simulink library "MCHP_Blockset"  (Simulink 7.5)
settings: Solver=ode45  SolverMode=SingleTasking  StartTime=0.0  StopTime=10.0  RelTol=1e-3
InitFcn:
  | disp('MCHP_Blockset_Library_InitFunction');
undefined symbols (not defined in the file): A0, A2, AD0, AVdd, B1, B5, B9, C10, C2, CMP2A, CMP3A, CMP4A, EXTREF1, EXTREF2, gcbh, MaxPer, MCHP_ACC_SAMx_Callback, MCHP_ADC_Callback, MCHP_ADC_HighSpeed_SAR_Callback, MCHP_ADC_HighSpeed_SAR_dsPIC_Callback, MCHP_ADC_SAME5x_Callback, MCHP_AFEC_SAM7x_Callback, MCHP_BUS_I2C_MASTER_callback, MCHP_BUS_SPI_callback, MCHP_C_function_Call_callback, MCHP_CN_Callback, MCHP_COMPARATOR1_callback, MCHP_CompilerOptimisation_Callback, MCHP_DACC_SAMx_Callback, MCHP_Digital_Input_Callback, MCHP_Digital_Output_Read_Callback, MCHP_Digital_Output_Write_Callback, MCHP_Fun, MCHP_HighSpeed_AnalogComparator_Callback, MCHP_IC_Callback, MCHP_IdleTask_Callback, MCHP_Interrupt_Callback, MCHP_Master_Callback, MCHP_MCPWM_Callback, MCHP_MCU_LOAD_Callback, MCHP_MCU_OVERLOAD_Callback, MCHP_MSI_Callback, MCHP_OC_HW_Callback, MCHP_OC_SW_Callback, MCHP_OP_AMP_Callback, MCHP_OrderInOut, MCHP_PDEC_Callback, MCHP_PGA_Callback, MCHP_PWM_Callback, MCHP_PWM_HighSpeed_Override_Callback, MCHP_PWM_HS_FEP_Callback, MCHP_PWM_SAM7x_Callback, MCHP_PWM_SAM7x_Override_Callback, MCHP_QDEC_SAMx_Callback, MCHP_QEI_Callback, MCHP_Scheduler_Options_Callback, MCHP_SECONDARY_CORE_Callback, MCHP_Tasks_State_Callback, MCHP_TCC_PWM_Callback, MCHP_TIMER_Config_Callback ... (+18)
libraries: MCHP_Blockset x2
(part 2 of 9)

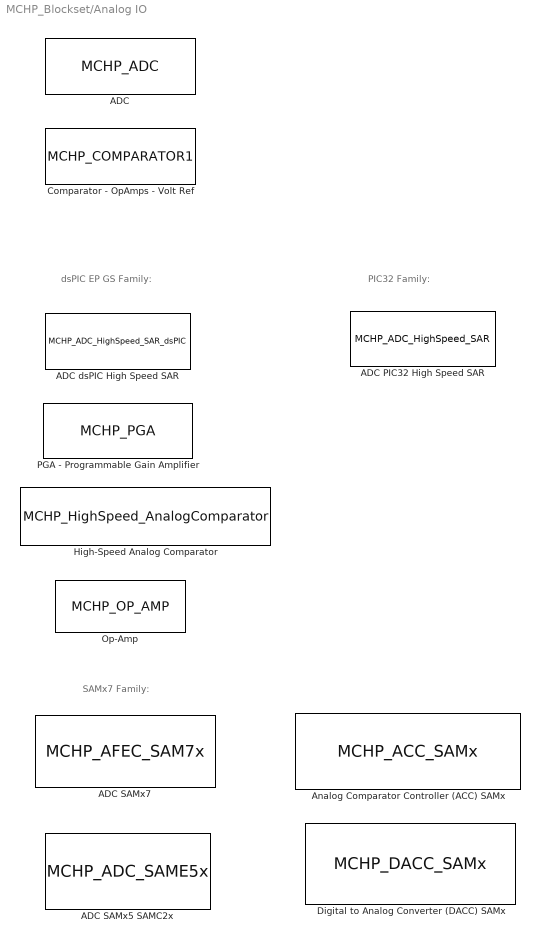
== system MCHP_Blockset/Analog IO ==
  note: dsPIC EP GS Family:
  note: PIC32 Family:
  note: SAMx7 Family:
  ADC : S-Function  Priority=5  InitFcn=MCHP_ADC_Callback(gcbh,'InitFcn');  FunctionName=MCHP_ADC  Parameters=SampleTime,[],MCHP_ADC_Callback(gcbh,'OutputType'),[],MCHP_ADC_Callback(gcbh,'OutputSize')  EnableBusSupport=off  mask{ADC_REF=1, Mode=10 bits (allows exact simultaneous sampling), FORM=0000 dddd dddd dddd ==> Unsigned integer, ADC_R=< 5    kOhm, nSAMPLECHANNELS=CH0 only, nSAMPLECHANNELS_12bits=CH0 only, SIMULTANEOUS=Simultaneously on all Channels, ADxCSS=[1 2], MUXA_CH0N=off, MUXA_CH123=Dynamic Options, MUXA_CH123_TXT=0, MUXB_CH0=AN1, MUXB_CH0N=on, MUXB_CH123=Dynamic Options, MUXB_CH123_TXT=0, SequenceRepeat=1, SequenceTiming=are done as fast as possible at end of previous time step, SSRC_SSRCG=Dynamic Options, SSRC_SSRCG_TXT=0, Update_BlockOutput=After all trig and conversion sequence, Trig_TimeStep=with each update of the ADC block output, ADC_DMA_CHANNEL=Use Interrupt instead of DMA, SampleTime=-1, Info=, MCHP_PORT=, MCHP_MASTERLINK=Testing_MasterBlock/Microchip Master, ADC_TIMING=0}
      mask prompts: ADC_REF "ADC"; FORM "Output Format"; ADC_R "Input Impedance"; nSAMPLECHANNELS "Sample and Hold Capacitor, and Sequences :"; nSAMPLECHANNELS_12bits "1 or 2 Sequences"; SIMULTANEOUS "Sampling happend:"; ADxCSS "CH0 Sequential Sampling, ex: [0 1 4 6] for AN0, AN1, AN4 and AN6"; MUXA_CH0N "Substract AN1 to CH0 (CH0 - AN1)"; MUXA_CH123 "CH1 : CH2 : CH3"; MUXB_CH0 "CH0 (B)"; MUXB_CH0N "Substract AN1 to CH0 (CH0 - AN1) (B)"; MUXB_CH123 "CH1 : CH2 : CH3 (B)"; SequenceRepeat "Repeat conversion sequence xx times"; SequenceTiming "Samples and Conversions"; SSRC_SSRCG "Trigger"; SSRC_SSRCG_TXT "Trigger SSRC_SSRCG value"; Update_BlockOutput "Update block output"; Trig_TimeStep "Trig Time Step"; ADC_DMA_CHANNEL "DMA"; SampleTime "Block Sample Time"
      mask init:
      | MCHP_ADC_Callback(gcbh,'INITIALISATION');
      settings: CopyFcn=MCHP_ADC_Callback(gcbh,'INITIALISATION');  PreSaveFcn=MCHP_ADC_Callback(gcbh,'InitFcn');MCHP_Fun.PreSaveFcn_DynamicOptions(gcbh);  OpenFcn=MCHP_ADC_Callback(gcbh,'OPEN');
      mask StyleString: popup(1),popup(10 bits (allows exact simultaneous sampling)|12 bits),popup(0000 dddd dddd dddd ==> Unsigned integer|ssss sddd dddd dddd ==> Signed integer|dddd dddd dddd 0000 ==> Unsigned fractional|sddd dddd dddd 0000  ==> Signed fractional),popup(< 100 Ohm|< 200 Ohm|< 500 Ohm|< 1    kOhm|< 2    kOhm|< 5    kOhm|< 10   kOhm|< 20   kOhm|< 50   kOhm|< 100  kOhm|< 200  kOhm|< 500  kOhm|< 1000 kOhm|max sampling time),popup(CH0 only|CH0 : CH1|CH0 : CH1 : CH2 : CH3|CH0 two sequences (A & B)|CH0 : CH1 two sequences (A & B)|CH0 : CH1 : CH2 : CH3 two seq (A & B)),popup(CH0 only|CH0 two sequences (A & B)),popup(Simultaneously on all Channels|in Sequence),edit,checkbox,popup(Dynamic Options),edit,popup(AN0|AN1|AN2|AN3|AN4|AN5|AN6|AN7|AN8|AN9|AN10|AN11|AN12|AN13|AN14|AN15|AN16|AN17|AN18|AN19|AN20|AN21|AN22|AN23|AN24|AN25|AN26|AN27|AN28|AN29|AN30|AN31|AN32|AN33|AN34|AN35|AN36|AN37|AN38|AN39|AN40|AN41|AN42|AN43|AN44|AN45|AN46|AN47|AN48|AN49|AN50|AN51|AN52|AN53|AN54|AN55|AN56|AN57|AN58|AN59|AN60|AN61|AN62|AN63|AN64|AN65|AN66|AN67|AN68|AN69|AN70|AN71|AN72|AN73|AN74|AN75|AN76|AN77|AN78|AN79|AN80|AN81|AN82|AN83|AN84|AN85|AN86|AN87|AN88|AN89|AN90|AN91|AN92|AN93|AN94|AN95|AN96|AN97|AN98|AN99|OA1|OA2|OA3|OA4|OA4),checkbox,popup(Dynamic Options),edit,edit,popup(are done as fast as possible at end of previous time step|are done as fast as possible ; triggered by user define source|are stretcheded to fit exactly previous time step|are continuously sampling as fast as possible),popup(Dynamic Options),edit,popup(After all trig and conversion sequence|After each trig and conversion sequence),popup(with each update of the ADC block output|not synchronised with ADC [timer based...]),popup(Use Interrupt instead of DMA|use DMA Channel 0|use DMA Channel 1|use DMA Channel 2|use DMA Channel 3|use DMA Channel 4|use DMA Channel 5|use DMA Channel 6|use DMA Channel 7|use DMA Channel 8|use DMA Channel 9|use DMA Channel 10|use DMA Channel 11|use DMA Channel 12|use DMA Channel 13|use DMA Channel 14|use DMA Channel 15),edit,edit,edit,edit,edit
      mask CallbackString: |MCHP_ADC_Callback(gcbh,'Mode');||MCHP_ADC_Callback(gcbh,'ADC_R');|MCHP_ADC_Callback(gcbh,'nSAMPLECHANNELS');|MCHP_ADC_Callback(gcbh,'nSAMPLECHANNELS_12bits');|MCHP_ADC_Callback(gcbh,'SIMULTANEOUS');|MCHP_ADC_Callback(gcbh,'ADxCSS');|MCHP_ADC_Callback(gcbh,'MUXA_CH0N');|MCHP_ADC_Callback(gcbh,'MUXA_CH123');||MCHP_ADC_Callback(gcbh,'MUXA_CH123');|MCHP_ADC_Callback(gcbh,'MUXA_CH123');||||MCHP_ADC_Callback(gcbh,'SequenceTiming');|||MCHP_ADC_Callback(gcbh,'Update_BlockOutput');|||||||
      mask TabNameString: ADC,ADC,ADC,ADC,ADC,ADC,ADC,ADC,ADC,ADC,ADC,ADC,ADC,ADC,ADC,ADC,Trig and Time Step,Trig and Time Step,Trig and Time Step,Trig and Time Step,Trig and Time Step,ADC,ADC,ADC,ADC,ADC,ADC
      mask Display:
      | MCHP_DrawLogo;
      | fprintf('ADC 1');
      | port_label('output',1,'AN1');
      | port_label('output',2,'AN2');
  ADC PIC32 High Speed SAR : S-Function  InitFcn=MCHP_ADC_HighSpeed_SAR_Callback(gcbh,'InitFcn');  FunctionName=MCHP_ADC_HighSpeed_SAR  Parameters=MCHP_ADC_HighSpeed_SAR_Callback(gcbh,'S_INPUT'),MCHP_ADC_HighSpeed_SAR_Callback(gcbh,'S_OUTPUT'),MCHP_ADC_HighSpeed_SAR_Callback(gcbh,'S_INPUT_Size'),MCHP_ADC_HighSpeed_SAR_Callback(gcbh,'S_OUTPUT_Size'),MCHP_ADC_HighSpeed_SAR_Callback(gcbh,'S_ListCustomDatatype'),SampleTime,0  EnableBusSupport=off  mask(ADC PIC32 EF family){ADC_VrefH=AVdd (default), ADC_VrefL=AVss (default), ADC_FRACT=Integer (right aligned), DMA_Size=Single trigger - (no DMA), ADC_Synchronisation=Triggered at end of previous time step, ADC_Trig=Dynamic Options, ADC_Trig_TXT=INT0 External Interrupt, ADC_TrigTimeStep=on, ADC_TrigInfo=0, SampleTime=.001, S_INPUT=[], S_INPUT_Size=[], S_OUTPUT=[5  5], S_OUTPUT_Size=[1  1], S_ListCustomDatatype=S.S_ListCustomDatatype={};, MCHP_USER_INTERRUPTS=0, MCHP_PORT={Analog Input 0}{AN0}15:2:B0;{Analog Input 1}{AN1}15:2:B1;, MCHP_MASTERLINK=pic32MZ_UTB_PIC32EF_ADC_Dedicated_BlockSavedForLib/Microchip Master, MCHP_CRC=1857122, ADC_Info=Total Time = 1.12(us), ADC0_pin=Dynamic Options, ADC0_pin_TXT=AN0 / B0 / Pin[36], ADC0_R=< 200 Ohm, ADC0_res=12 bits, ADC0_signed=unsigned 16 bits, ADC0_FILTER=No Oversampling, ADC0_FILTER_nSamples=256 samples, ADC0_STRGEN=End sampling and start conversion, ADC0_SSAMPEN=off, ADC0_Info=tSmp_min=80(ns) x 0 = 0(s) ; tConv=560(ns) x 1 = 560(ns) ; TOTAL=560(ns), ADC1_pin=Dynamic Options, ADC1_pin_TXT=AN1 / B1 / Pin[35], ADC1_R=< 200 Ohm, ADC1_res=12 bits, ADC1_signed=unsigned 16 bits, ADC1_FILTER=No Oversampling, ADC1_FILTER_nSamples=256 samples, ADC1_STRGEN=End sampling and start conversion, ADC1_SSAMPEN=off, ADC1_Info=tSmp_min=80(ns) x 0 = 0(s) ; tConv=560(ns) x 1 = 560(ns) ; TOTAL=560(ns), ADC2_pin=Dynamic Options, ADC2_pin_TXT=Not used, ADC2_R=< 200 Ohm, ADC2_res=12 bits, ADC2_signed=unsigned 16 bits, ADC2_FILTER=No Oversampling, ADC2_FILTER_nSamples=256 samples, ADC2_STRGEN=End sampling and start conversion, ADC2_SSAMPEN=off, ADC2_Info=tSmp_min=40(ns) x -2 = -80(ns) ; tConv=240(ns) x -1 = -240(ns) ; TOTAL=-240(ns), ADC3_pin=Dynamic Options, ADC3_pin_TXT=Not used, ADC3_R=< 200 Ohm, ADC3_res=12 bits, ADC3_signed=unsigned 16 bits, ADC3_FILTER=No Oversampling, ADC3_FILTER_nSamples=256 samples, ADC3_STRGEN=End sampling and start conversion, ADC3_SSAMPEN=off, ADC3_Info=tSmp_min=40(ns) x -2 = -80(ns) ; tConv=240(ns) x -1 = -240(ns) ; TOTAL=-240(ns), ADC4_pin=Dynamic Options, ADC4_pin_TXT=Not used, ADC4_R=< 200 Ohm, ADC4_res=12 bits, ADC4_signed=unsigned 16 bits, ADC4_FILTER=No Oversampling, ADC4_FILTER_nSamples=256 samples, ADC4_STRGEN=End sampling and start conversion, ADC4_SSAMPEN=off, ADC4_Info=tSmp_min=40(ns) x -2 = -80(ns) ; tConv=240(ns) x -1 = -240(ns) ; TOTAL=-240(ns), ADC5_pin=Dynamic Options, ADC5_pin_TXT=Not used, ADC5_R=< 200 Ohm, ADC5_res=12 bits, ADC5_signed=unsigned 16 bits, ADC5_FILTER=Burst convert of n samples are Summed, ADC5_FILTER_nSamples=256 samples, ADC5_STRGEN=End sampling and start conversion, ADC5_SSAMPEN=on, ADC5_Info=tSmp_min=40(ns) x -2 = -80(ns) ; tConv=240(ns) x -1 = -240(ns) ; TOTAL=-240(ns), ADC6_pin=Dynamic Options, ADC6_pin_TXT=Not used, ADC6_R=< 200 Ohm, ADC6_res=12 bits, ADC6_signed=unsigned 16 bits, ADC6_FILTER=Burst convert of n samples are Summed, ADC6_FILTER_nSamples=256 samples, ADC6_STRGEN=End sampling and start conversion, ADC6_SSAMPEN=on, ADC6_Info=tSmp_min=40(ns) x -2 = -80(ns) ; tConv=240(ns) x -1 = -240(ns) ; TOTAL=-240(ns), ADC7_R=< 200 Ohm, ADC7_res=12 bits, ADC7_AN0=Not used, ADC7_AN1=Not used, ADC7_AN2=Not used, ADC7_AN3=Not used, ADC7_AN4=Not used, ADC7_AN5=Not used, ADC7_AN6=Not used, ADC7_AN7=Not used, ADC7_AN8=Not used, ADC7_AN9=Not used, ADC7_AN10=Not used, ADC7_AN11=Not used, ADC7_AN12=Not used, ADC7_AN13=Not used, ADC7_AN14=Not used, ADC7_AN15=Not used, ADC7_AN16=Not used, ADC7_AN17=Not used, ADC7_AN18=Not used, ADC7_AN19=Not used, ADC7_AN20=Not used, ADC7_AN21=Not used, ADC7_AN22=Not used, ADC7_AN23=Not used, ADC7_AN24=Not used, ADC7_AN25=Not used, ADC7_AN26=Not used, ADC7_AN27=Not used, ADC7_AN28=Not used, ADC7_AN29=Not used, ADC7_AN30=Not used, ADC7_AN31=Not used, ADC7_AN32=Not used, ADC7_AN33=Not used, ADC7_AN34=Not used, ADC7_AN35=Not used, ADC7_AN36=Not used, ADC7_AN37=Not used, ADC7_AN38=Not used, ADC7_AN39=Not used, ADC7_AN40=Not used, ADC7_AN41=Not used, ADC7_AN42=Not used, ADC7_AN43=Not used, ADC7_AN44=Not used, ADC7_AN45=Not used, ADC7_AN46=Not used, ADC7_AN47=Not used, ADC7_AN48=Not used, ADC7_AN49=Not used, ADC7_AN50=Not used, ADC7_AN51=Not used, ADC7_AN52=Not used, ADC7_AN53=Not used, ADC7_AN54=Not used, ADC7_AN55=Not used, ADC7_AN56=Not used, ADC7_AN57=Not used, ADC7_AN58=Not used, ADC7_AN59=Not used, ADC7_AN60=Not used, ADC7_AN61=Not used, ADC7_AN62=Not used, ADC7_AN63=Not used, CTMU_Temp=Not used, Vbat=Not used, IVref=Not used, IVTemp=Not used}
      mask prompts: ADC_VrefH "Positive reference voltage (vref H)"; ADC_VrefL "Negative reference voltage (verf L)"; ADC_FRACT "Conversion Format (Global to all ADC blocks)"; DMA_Size "Multiple trigger - Vector output - for ADC[0-6] of current block"; ADC_Synchronisation "ADC Sample and Conversion"; ADC_Trig "User defined trigger:"; ADC_TrigTimeStep "The model base Time Step is triggered by the the last ADC conversion using this trigger"; ADC_TrigInfo "ADC Trigger Info"; SampleTime "Block output sample time"; ADC_Info "Infos"; ADC0_pin "Analog input pin"; ADC0_R "Input Impedance"; ADC0_res "Resolution of conversion"; ADC0_signed "Output format"; ADC0_FILTER "Filter / Oversampling"; ADC0_FILTER_nSamples "Filter / Oversampling burst of:"; ADC0_STRGEN "Initial trigger option:"; ADC0_SSAMPEN "Ensure synchronous sampling (might add a delay)"; ADC0_Info "ADC0 !Info"; ADC1_pin "Analog input pin"; ADC1_pin_TXT "ADC0_pin_TXT"; ADC1_R "Input Impedance"; ADC1_res "Resolution of conversion"; ADC1_signed "Output format"; ADC1_FILTER "Filter / Oversampling"; ADC1_FILTER_nSamples "Filter / Oversampling burst of:"; ADC1_STRGEN "Initial trigger option:"; ADC1_SSAMPEN "Ensure synchronous sampling (might add a delay)"; ADC1_Info "ADC1 Infos"; ADC2_pin "Analog input pin"; ADC2_R "Input Impedance"; ADC2_res "Resolution of conversion"; ADC2_signed "Output format"; ADC2_FILTER "Filter / Oversampling"; ADC2_FILTER_nSamples "Filter / Oversampling burst of:"; ADC2_STRGEN "Initial trigger option:"; ADC2_SSAMPEN "Ensure synchronous sampling (might add a delay)"; ADC2_Info "ADC2 Infos"; ADC3_pin "Analog input pin"; ADC3_R "Input Impedance"; ADC3_res "Resolution of conversion"; ADC3_signed "Output format"; ADC3_FILTER "Filter / Oversampling"; ADC3_FILTER_nSamples "Filter / Oversampling burst of:"; ADC3_STRGEN "Initial trigger option:"; ADC3_SSAMPEN "Ensure synchronous sampling (might add a delay)"; ADC3_Info "ADC3 Infos"; ADC4_pin "Analog input pin"; ADC4_R "Input Impedance"; ADC4_res "Resolution of conversion"; ADC4_signed "Output format"; ADC4_FILTER "Filter / Oversampling"; ADC4_FILTER_nSamples "Filter / Oversampling burst of:"; ADC4_STRGEN "Initial trigger option:"; ADC4_SSAMPEN "Ensure synchronous sampling (might add a delay)"; ADC4_Info "ADC4 Infos"; ADC5_pin "Analog input pin"; ADC5_R "Input Impedance"; ADC5_res "Resolution of conversion"; ADC5_signed "Output format"; ADC5_FILTER "Filter / Oversampling"; ADC5_FILTER_nSamples "Filter / Oversampling burst of:"; ADC5_STRGEN "Initial trigger option:"; ADC5_SSAMPEN "Ensure synchronous sampling (might add a delay)"; ADC5_Info "ADC5 Infos"; ADC6_pin "Analog input pin"; ADC6_R "Input Impedance"; ADC6_res "Resolution of conversion"; ADC6_signed "Output format"; ADC6_FILTER "Filter / Oversampling"; ADC6_FILTER_nSamples "Filter / Oversampling burst of:"; ADC6_STRGEN "Initial trigger option:"; ADC6_SSAMPEN "Ensure synchronous sampling (might add a delay)"; ADC6_Info "ADC6 Infos"; ADC7_R "ADC7 Input Impedance (Class 2 and 3 inputs)"; ADC7_res "ADC7 Resolution of conversion (Class 2 and 3 inputs)"; ADC7_AN0 "AN0 pin"; ADC7_AN1 "AN1 pin"; ADC7_AN2 "AN2_pin"; ADC7_AN3 "AN3_pin"; ADC7_AN4 ""; ADC7_AN5 ""; ADC7_AN6 ""; ADC7_AN7 ""; ADC7_AN8 ""; ADC7_AN9 ""; ADC7_AN10 ""; ADC7_AN11 ""; ADC7_AN12 ""; ADC7_AN13 ""; ADC7_AN14 ""; ADC7_AN15 ""; ADC7_AN16 ""; ADC7_AN17 ""; ADC7_AN18 ""; ADC7_AN19 ""; ADC7_AN20 ""; ADC7_AN21 ""; ADC7_AN22 ""; ADC7_AN23 ""; ADC7_AN24 ""; ADC7_AN25 ""; ADC7_AN26 ""; ADC7_AN27 ""; ADC7_AN28 ""; ADC7_AN29 ""; ADC7_AN30 ""; ADC7_AN31 ""; ADC7_AN32 ""; ADC7_AN33 ""; ADC7_AN34 ""; ADC7_AN35 ""; ADC7_AN36 ""; ADC7_AN37 ""; ADC7_AN38 ""; ADC7_AN39 ""; ADC7_AN40 ""; ADC7_AN41 ""; ADC7_AN42 ""; ADC7_AN43 ""; ADC7_AN44 ""; ADC7_AN45 ""; ADC7_AN46 ""; ADC7_AN47 ""; ADC7_AN48 ""; ADC7_AN49 ""; ADC7_AN50 ""; ADC7_AN51 ""; ADC7_AN52 ""; ADC7_AN53 ""; ADC7_AN54 ""; ADC7_AN55 ""; ADC7_AN56 ""; ADC7_AN57 ""; ADC7_AN58 ""; ADC7_AN59 ""; ADC7_AN60 ""; ADC7_AN61 ""; ADC7_AN62 ""; ADC7_AN63 ""; CTMU_Temp "CTMU Temp"; Vbat "Vbat / 2"; IVref "Vref (1.2V)"; IVTemp "Temp"
      mask init:
      | MCHP_ADC_HighSpeed_SAR_Callback(gcbh,'INITIALISATION');
      settings: CopyFcn=MCHP_ADC_HighSpeed_SAR_Callback(gcbh,'CopyFcn');  PreSaveFcn=MCHP_Fun.PreSaveFcn_DynamicOptions(gcbh);  OpenFcn=MCHP_ADC_HighSpeed_SAR_Callback(gcbh,'OPEN');
      mask StyleString: popup(AVdd (default)|Vref +),popup(AVss (default)|Vref -),popup(Integer (right aligned)|Fractional (left aligned)),popup(Single trigger - (no DMA)|1 trig / 1 element output (use DMA ping-pong buffer)|2 trig / 2 elements output (use DMA ping-pong buffer)|4 trig / 4 elements output (use DMA ping-pong buffer)|8 trig / 8 elements output (use DMA ping-pong buffer)|16 trig / 16 elements output (use DMA ping-pong buffer)|32 trig / 32 elements output (use DMA ping-pong buffer)|64 trig / 64 elements output (use DMA ping-pong buffer)|128 trig / 128 elements output (use DMA ping-pong buffer)),popup(Triggered at end of previous time step|Triggered by custom source|Continuously triggered. Output is last conversion),popup(Dynamic Options),edit,checkbox,edit,edit,edit,edit,edit,edit,edit,edit,edit,edit,edit,edit,popup(Dynamic Options),edit,popup(< 200 Ohm|< 500 Ohm|< 1    kOhm|< 2    kOhm|< 5    kOhm|< 10   kOhm|< 20   kOhm|< 50   kOhm|< 100  kOhm|< 200  kOhm|< 500  kOhm|max sampling time),popup(12 bits|10 bits|8 bits|6 bits),popup(unsigned 32 bits (native)|signed 32 bits (native)|unsigned 16 bits|signed 16 bits),popup(No Oversampling|Burst convert of n samples are Summed|Burst convert of n samples are Averaged),popup(2 samples|4 samples|8 samples|16 samples|32 samples|64 samples|128 samples|256 samples),popup(End sampling and start conversion|Start sampling followed by conversion),checkbox,edit,popup(Dynamic Options),edit,popup(< 200 Ohm|< 500 Ohm|< 1    kOhm|< 2    kOhm|< 5    kOhm|< 10   kOhm|< 20   kOhm|< 50   kOhm|< 100  kOhm|< 200  kOhm|< 500  kOhm|max sampling time),popup(12 bits|10 bits|8 bits|6 bits),popup(unsigned 32 bits (native)|signed 32 bits (native)|unsigned 16 bits|signed 16 bits),popup(No Oversampling|Burst convert of n samples are Summed|Burst convert of n samples are Averaged),popup(2 samples|4 samples|8 samples|16 samples|32 samples|64 samples|128 samples|256 samples),popup(End sampling and start conversion|Start sampling followed by conversion),checkbox,edit,popup(Dynamic Options),edit,popup(< 200 Ohm|< 500 Ohm|< 1    kOhm|< 2    kOhm|< 5    kOhm|< 10   kOhm|< 20   kOhm|< 50   kOhm|< 100  kOhm|< 200  kOhm|< 500  kOhm|max sampling time),popup(12 bits|10 bits|8 bits|6 bits),popup(unsigned 32 bits (native)|signed 32 bits (native)|unsigned 16 bits|signed 16 bits),popup(No Oversampling|Burst convert of n samples are Summed|Burst convert of n samples are Averaged),popup(2 samples|4 samples|8 samples|16 samples|32 samples|64 samples|128 samples|256 samples),popup(End sampling and start conversion|Start sampling followed by conversion),checkbox,edit,popup(Dynamic Options),edit,popup(< 200 Ohm|< 500 Ohm|< 1    kOhm|< 2    kOhm|< 5    kOhm|< 10   kOhm|< 20   kOhm|< 50   kOhm|< 100  kOhm|< 200  kOhm|< 500  kOhm|max sampling time),popup(12 bits|10 bits|8 bits|6 bits),popup(unsigned 32 bits (native)|signed 32 bits (native)|unsigned 16 bits|signed 16 bits),popup(No Oversampling|Burst convert of n samples are Summed|Burst convert of n samples are Averaged),popup(2 samples|4 samples|8 samples|16 samples|32 samples|64 samples|128 samples|256 samples),popup(End sampling and start conversion|Start sampling followed by conversion),checkbox,edit,popup(Dynamic Options),edit,popup(< 200 Ohm|< 500 Ohm|< 1    kOhm|< 2    kOhm|< 5    kOhm|< 10   kOhm|< 20   kOhm|< 50   kOhm|< 100  kOhm|< 200  kOhm|< 500  kOhm|max sampling time),popup(12 bits|10 bits|8 bits|6 bits),popup(unsigned 32 bits (native)|signed 32 bits (native)|unsigned 16 bits|signed 16 bits),popup(No Oversampling|Burst convert of n samples are Summed|Burst convert of n samples are Averaged),popup(2 samples|4 samples|8 samples|16 samples|32 samples|64 samples|128 samples|256 samples),popup(End sampling and start conversion|Start sampling followed by conversion),checkbox,edit,popup(Dynamic Options),edit,popup(< 200 Ohm|< 500 Ohm|< 1    kOhm|< 2    kOhm|< 5    kOhm|< 10   kOhm|< 20   kOhm|< 50   kOhm|< 100  kOhm|< 200  kOhm|< 500  kOhm|max sampling time),popup(12 bits|10 bits|8 bits|6 bits),popup(unsigned 32 bits (native)|signed 32 bits (native)|unsigned 16 bits|signed 16 bits),popup(No Oversampling|Burst convert of n samples are Summed|Burst convert of n samples are Averaged),popup(2 samples|4 samples|8 samples|16 samples|32 samples|64 samples|128 samples|256 samples),popup(End sampling and start conversion|Start sampling followed by conversion),checkbox,edit,popup(Dynamic Options),edit,popup(< 200 Ohm|< 500 Ohm|< 1    kOhm|< 2    kOhm|< 5    kOhm|< 10   kOhm|< 20   kOhm|< 50   kOhm|< 100  kOhm|< 200  kOhm|< 500  kOhm|max sampling time),popup(12 bits|10 bits|8 bits|6 bits),popup(unsigned 32 bits (native)|signed 32 bits (native)|unsigned 16 bits|signed 16 bits),popup(No Oversampling|Burst convert of n samples are Summed|Burst convert of n samples are Averaged),popup(2 samples|4 samples|8 samples|16 samples|32 samples|64 samples|128 samples|256 samples),popup(End sampling and start conversion|Start sampling followed by conversion),checkbox,edit,popup(< 200 Ohm|< 500 Ohm|< 1    kOhm|< 2    kOhm|< 5    kOhm|< 10   kOhm|< 20   kOhm|< 50   kOhm|< 100  kOhm|< 200  kOhm|< 500  kOhm|max sampling time),popup(12 bits|10 bits|8 bits|6 bits),popup(Not used|unsigned int16 |signed int16|unsigned int32|signed int32|---BurstSample with internal Digital filter---|2 samples averaged - unsigned int16|4 samples averaged - unsigned int16|8 samples averaged - unsigned int16|16 samples averaged - unsigned int16|32 samples averaged - unsigned int16|64 samples averaged - unsigned int16|128 samples averaged - unsigned int16|256 samples averaged - unsigned int16|---|2 samples averaged - signed int16|4 samples averaged - signed int16|8 samples averaged - signed int16|16 samples averaged - signed int16|32 samples averaged - signed int16|64 samples averaged - signed int16|128 samples averaged - signed int16|256 samples averaged - signed int16|---|4 samples summed - unsigned int16|8 samples summed - unsigned int16|16 samples summed - unsigned int16|32 samples summed - unsigned int16|64 samples summed - unsigned int16|128 samples summed - unsigned int16|256 samples summed - unsigned int16|---|2 samples summed - signed int16|4 samples summed - signed int16|8 samples summed - signed int16|16 samples summed - signed int16|32 samples summed - signed int16|64 samples summed - signed int16|128 samples summed - signed int16|256 samples summed - signed int16|---|2 samples averaged - unsigned int32|4 samples averaged - unsigned int32|8 samples averaged - unsigned int32|16 samples averaged - unsigned int32|32 samples averaged - unsigned int32|64 samples averaged - unsigned int32|128 samples averaged - unsigned int32|256 samples averaged - unsigned int32|---|2 samples averaged - signed int32|4 samples averaged - signed int32|8 samples averaged - signed int32|16 samples averaged - signed int32|32 samples averaged - signed int32|64 samples averaged - signed int32|128 samples averaged - signed int32|256 samples averaged - signed int32|---|4 samples summed - unsigned int32|8 samples summed - unsigned int32|16 samples summed - unsigned int32|32 samples summed - unsigned int32|64 samples summed - unsigned int32|128 samples summed - unsigned int32|256 samples summed - unsigned int32|---|2 samples summed - signed int32|4 samples summed - signed int32|8 samples summed - signed int32|16 samples summed - signed int32|32 samples summed - signed int32|64 samples summed - signed int32|128 samples summed - signed int32|256 samples summed - signed int32),popup(Not used|unsigned int16 |signed int16|unsigned int32|signed int32|---BurstSample with internal Digital filter---|2 samples averaged - unsigned int16|4 samples averaged - unsigned int16|8 samples averaged - unsigned int16|16 samples averaged - unsigned int16|32 samples averaged - unsigned int16|64 samples averaged - unsigned int16|128 samples averaged - unsigned int16|256 samples averaged - unsigned int16|---|2 samples averaged - signed int16|4 samples averaged - signed int16|8 samples averaged - signed int16|16 samples averaged - signed int16|32 samples averaged - signed int16|64 samples averaged - signed int16|128 samples averaged - signed int16|256 samples averaged - signed int16|---|4 samples summed - unsigned int16|8 samples summed - unsigned int16|16 samples summed - unsigned int16|32 samples summed - unsigned int16|64 samples summed - unsigned int16|128 samples summed - unsigned int16|256 samples summed - unsigned int16|---|2 samples summed - signed int16|4 samples summed - signed int16|8 samples summed - signed int16|16 samples summed - signed int16|32 samples summed - signed int16|64 samples summed - signed int16|128 samples summed - signed int16|256 samples summed - signed int16|---|2 samples averaged - unsigned int32|4 samples averaged - unsigned int32|8 samples averaged - unsigned int32|16 samples averaged - unsigned int32|32 samples averaged - unsigned int32|64 samples averaged - unsigned int32|128 samples averaged - unsigned int32|256 samples averaged - unsigned int32|---|2 samples averaged - signed int32|4 samples averaged - signed int32|8 samples averaged - signed int32|16 samples averaged - signed int32|32 samples averaged - signed int32|64 samples averaged - signed int32|128 samples averaged - signed int32|256 samples averaged - signed int32|---|4 samples summed - unsigned int32|8 samples summed - unsigned int32|16 samples summed - unsigned int32|32 samples summed - unsigned int32|64 samples summed - unsigned int32|128 samples summed - unsigned int32|256 samples summed - unsigned int32|---|2 samples summed - signed int32|4 samples summed - signed int32|8 samples summed - signed int32|16 samples summed - signed int32|32 samples summed - signed int32|64 samples summed - signed int32|128 samples summed - signed int32|256 samples summed - signed int32),popup(Not used|unsigned int16 |signed int16|unsigned int32|signed int32|---BurstSample with internal Digital filter---|2 samples averaged - unsigned int16|4 samples averaged - unsigned int16|8 samples averaged - unsigned int16|16 samples averaged - unsigned int16|32 samples averaged - unsigned int16|64 samples averaged - unsigned int16|128 samples averaged - unsigned int16|256 samples averaged - unsigned int16|---|2 samples averaged - signed int16|4 samples averaged - signed int16|8 samples averaged - signed int16|16 samples averaged - signed int16|32 samples averaged - signed int16|64 samples averaged - signed int16|128 samples averaged - signed int16|256 samples averaged - signed int16|---|4 samples summed - unsigned int16|8 samples summed - unsigned int16|16 samples summed - unsigned int16|32 samples summed - unsigned int16|64 samples summed - unsigned int16|128 samples summed - unsigned int16|256 samples summed - unsigned int16|---|2 samples summed - signed int16|4 samples summed - signed int16|8 samples summed - signed int16|16 samples summed - signed int16|32 samples summed - signed int16|64 samples summed - signed int16|128 samples summed - signed int16|256 samples summed - signed int16|---|2 samples averaged - unsigned int32|4 samples averaged - unsigned int32|8 samples averaged - unsigned int32|16 samples averaged - unsigned int32|32 samples averaged - unsigned int32|64 samples averaged - unsigned int32|128 samples averaged - unsigned int32|256 samples averaged - unsigned int32|---|2 samples averaged - signed int32|4 samples averaged - signed int32|8 samples averaged - signed int32|16 samples averaged - signed int32|32 samples averaged - signed int32|64 samples averaged - signed int32|128 samples averaged - signed int32|256 samples averaged - signed int32|---|4 samples summed - unsigned int32|8 samples summed - unsigned int32|16 samples summed - unsigned int32|32 samples summed - unsigned int32|64 samples summed - unsigned int32|128 samples summed - unsigned int32|256 samples summed - unsigned int32|---|2 samples summed - signed int32|4 samples summed - signed int32|8 samples summed - signed int32|16 samples summed - signed int32|32 samples summed - signed int32|64 samples summed - signed int32|128 samples summed - signed int32|256 samples summed - signed int32),popup(Not used|unsigned int16 |signed int16|unsigned int32|signed int32|---BurstSample with internal Digital filter---|2 samples averaged - unsigned int16|4 samples averaged - unsigned int16|8 samples averaged - unsigned int16|16 samples averaged - unsigned int16|32 samples averaged - unsigned int16|64 samples averaged - unsigned int16|128 samples averaged - unsigned int16|256 samples averaged - unsigned int16|---|2 samples averaged - signed int16|4 samples averaged - signed int16|8 samples averaged - signed int16|16 samples averaged - signed int16|32 samples averaged - signed int16|64 samples averaged - signed int16|128 samples averaged - signed int16|256 samples averaged - signed int16|---|4 samples summed - unsigned int16|8 samples summed - unsigned int16|16 samples summed - unsigned int16|32 samples summed - unsigned int16|64 samples summed - unsigned int16|128 samples summed - unsigned int16|256 samples summed - unsigned int16|---|2 samples summed - signed int16|4 samples summed - signed int16|8 samples summed - signed int16|16 samples summed - signed int16|32 samples summed - signed int16|64 samples summed - signed int16|128 samples summed - signed int16|256 samples summed - signed int16|---|2 samples averaged - unsigned int32|4 samples averaged - unsigned int32|8 samples averaged - unsigned int32|16 samples averaged - unsigned int32|32 samples averaged - unsigned int32|64 samples averaged - unsigned int32|128 samples averaged - unsigned int32|256 samples averaged - unsigned int32|---|2 samples averaged - signed int32|4 samples averaged - signed int32|8 samples averaged - signed int32|16 samples averaged - signed int32|32 samples averaged - signed int32|64 samples averaged - signed int32|128 samples averaged - signed int32|256 samples averaged - signed int32|---|4 samples summed - unsigned int32|8 samples summed - unsigned int32|16 samples summed - unsigned int32|32 samples summed - unsigned int32|64 samples summed - unsigned int32|128 samples summed - unsigned int32|256 samples summed - unsigned int32|---|2 samples summed - signed int32|4 samples summed - signed int32|8 samples summed - signed int32|16 samples summed - signed int32|32 samples summed - signed int32|64 samples summed - signed int32|128 samples summed - signed int32|256 samples summed - signed int32),popup(Not used|unsigned int16 |signed int16|unsigned int32|signed int32|---BurstSample with internal Digital filter---|2 samples averaged - unsigned int16|4 samples averaged - unsigned int16|8 samples averaged - unsigned int16|16 samples averaged - unsigned int16|32 samples averaged - unsigned int16|64 samples averaged - unsigned int16|128 samples averaged - unsigned int16|256 samples averaged - unsigned int16|---|2 samples averaged - signed int16|4 samples averaged - signed int16|8 samples averaged - signed int16|16 samples averaged - signed int16|32 samples averaged - signed int16|64 samples averaged - signed int16|128 samples averaged - signed int16|256 samples averaged - signed int16|---|4 samples summed - unsigned int16|8 samples summed - unsigned int16|16 samples summed - unsigned int16|32 samples summed - unsigned int16|64 samples summed - unsigned int16|128 samples summed - unsigned int16|256 samples summed - unsigned int16|---|2 samples summed - signed int16|4 samples summed - signed int16|8 samples summed - signed int16|16 samples summed - signed int16|32 samples summed - signed int16|64 samples summed - signed int16|128 samples summed - signed int16|256 samples summed - signed int16|---|2 samples averaged - unsigned int32|4 samples averaged - unsigned int32|8 samples averaged - unsigned int32|16 samples averaged - unsigned int32|32 samples averaged - unsigned int32|64 samples averaged - unsigned int32|128 samples averaged - unsigned int32|256 samples averaged - unsigned int32|---|2 samples averaged - signed int32|4 samples averaged - signed int32|8 samples averaged - signed int32|16 samples averaged - signed int32|32 samples averaged - signed int32|64 samples averaged - signed int32|128 samples averaged - signed int32|256 samples averaged - signed int32|---|4 samples summed - unsigned int32|8 samples summed - unsigned int32|16 samples summed - unsigned int32|32 samples summed - unsigned int32|64 samples summed - unsigned int32|128 samples summed - unsigned int32|256 samples summed - unsigned int32|---|2 samples summed - signed int32|4 samples summed - signed int32|8 samples summed - signed int32|16 samples summed - signed int32|32 samples summed - signed int32|64 samples summed - signed int32|128 samples summed - signed int32|256 samples summed - signed int32),popup(Not used|unsigned int16 |signed int16|unsigned int32|signed int32|---BurstSample with internal Digital filter---|2 samples averaged - unsigned int16|4 samples averaged - unsigned int16|8 samples averaged - unsigned int16|16 samples averaged - unsigned int16|32 samples averaged - unsigned int16|64 samples averaged - unsigned int16|128 samples averaged - unsigned int16|256 samples averaged - unsigned int16|---|2 samples averaged - signed int16|4 samples averaged - signed int16|8 samples averaged - signed int16|16 samples averaged - signed int16|32 samples averaged - signed int16|64 samples averaged - signed int16|128 samples averaged - signed int16|256 samples averaged - signed int16|---|4 samples summed - unsigned int16|8 samples summed - unsigned int16|16 samples summed - unsigned int16|32 samples summed - unsigned int16|64 samples summed - unsigned int16|128 samples summed - unsigned int16|256 samples summed - unsigned int16|---|2 samples summed - signed int16|4 samples summed - signed int16|8 samples summed - signed int16|16 samples summed - signed int16|32 samples summed - signed int16|64 samples summed - signed int16|128 samples summed - signed int16|256 samples summed - signed int16|---|2 samples averaged - unsigned int32|4 samples averaged - unsigned int32|8 samples averaged - unsigned int32|16 samples averaged - unsigned int32|32 samples averaged - unsigned int32|64 samples averaged - unsigned int32|128 samples averaged - unsigned int32|256 samples averaged - unsigned int32|---|2 samples averaged - signed int32|4 samples averaged - signed int32|8 samples averaged - signed int32|16 samples averaged - signed int32|32 samples averaged - signed int32|64 samples averaged - signed int32|128 samples averaged - signed int32|256 samples averaged - signed int32|---|4 samples summed - unsigned int32|8 samples summed - unsigned int32|16 samples summed - unsigned int32|32 samples summed - unsigned int32|64 samples summed - unsigned int32|128 samples summed - unsigned int32|256 samples summed - unsigned int32|---|2 samples summed - signed int32|4 samples summed - signed int32|8 samples summed - signed int32|16 samples summed - signed int32|32 samples summed - signed int32|64 samples summed - signed int32|128 samples summed - signed int32|256 samples summed - signed int32),popup(Not used|unsigned int16 |signed int16|unsigned int32|signed int32|---BurstSample with internal Digital filter---|2 samples averaged - unsigned int16|4 samples averaged - unsigned int16|8 samples averaged - unsigned int16|16 samples averaged - unsigned int16|32 samples averaged - unsigned int16|64 samples averaged - unsigned int16|128 samples averaged - unsigned int16|256 samples averaged - unsigned int16|---|2 samples averaged - signed int16|4 samples averaged - signed int16|8 samples averaged - signed int16|16 samples averaged - signed int16|32 samples averaged - signed int16|64 samples averaged - signed int16|128 samples averaged - signed int16|256 samples averaged - signed int16|---|4 samples summed - unsigned int16|8 samples summed - unsigned int16|16 samples summed - unsigned int16|32 samples summed - unsigned int16|64 samples summed - unsigned int16|128 samples summed - unsigned int16|256 samples summed - unsigned int16|---|2 samples summed - signed int16|4 samples summed - signed int16|8 samples summed - signed int16|16 samples summed - signed int16|32 samples summed - signed int16|64 samples summed - signed int16|128 samples summed - signed int16|256 samples summed - signed int16|---|2 samples averaged - unsigned int32|4 samples averaged - unsigned int32|8 samples averaged - unsigned int32|16 samples averaged - unsigned int32|32 samples averaged - unsigned int32|64 samples averaged - unsigned int32|128 samples averaged - unsigned int32|256 samples averaged - unsigned int32|---|2 samples averaged - signed int32|4 samples averaged - signed int32|8 samples averaged - signed int32|16 samples averaged - signed int32|32 samples averaged - signed int32|64 samples averaged - signed int32|128 samples averaged - signed int32|256 samples averaged - signed int32|---|4 samples summed - unsigned int32|8 samples summed - unsigned int32|16 samples summed - unsigned int32|32 samples summed - unsigned int32|64 samples summed - unsigned int32|128 samples summed - unsigned int32|256 samples summed - unsigned int32|---|2 samples summed - signed int32|4 samples summed - signed int32|8 samples summed - signed int32|16 samples summed - signed int32|32 samples summed - signed int32|64 samples summed - signed int32|128 samples summed - signed int32|256 samples summed - signed int32),popup(Not used|unsigned int16 |signed int16|unsigned int32|signed int32|---BurstSample with internal Digital filter---|2 samples averaged - unsigned int16|4 samples averaged - unsigned int16|8 samples averaged - unsigned int16|16 samples averaged - unsigned int16|32 samples averaged - unsigned int16|64 samples averaged - unsigned int16|128 samples averaged - unsigned int16|256 samples averaged - unsigned int16|---|2 samples averaged - signed int16|4 samples averaged - signed int16|8 samples averaged - signed int16|16 samples averaged - signed int16|32 samples averaged - signed int16|64 samples averaged - signed int16|128 samples averaged - signed int16|256 samples averaged - signed int16|---|4 samples summed - unsigned int16|8 samples summed - unsigned int16|16 samples summed - unsigned int16|32 samples summed - unsigned int16|64 samples summed - unsigned int16|128 samples summed - unsigned int16|256 samples summed - unsigned int16|---|2 samples summed - signed int16|4 samples summed - signed int16|8 samples summed - signed int16|16 samples summed - signed int16|32 samples summed - signed int16|64 samples summed - signed int16|128 samples summed - signed int16|256 samples summed - signed int16|---|2 samples averaged - unsigned int32|4 samples averaged - unsigned int32|8 samples averaged - unsigned int32|16 samples averaged - unsigned int32|32 samples averaged - unsigned int32|64 samples averaged - unsigned int32|128 samples averaged - unsigned int32|256 samples averaged - unsigned int32|---|2 samples averaged - signed int32|4 samples averaged - signed int32|8 samples averaged - signed int32|16 samples averaged - signed int32|32 samples averaged - signed int32|64 samples averaged - signed int32|128 samples averaged - signed int32|256 samples averaged - signed int32|---|4 samples summed - unsigned int32|8 samples summed - unsigned int32|16 samples summed - unsigned int32|32 samples summed - unsigned int32|64 samples summed - unsigned int32|128 samples summed - unsigned int32|256 samples summed - unsigned int32|---|2 samples summed - signed int32|4 samples summed - signed int32|8 samples summed - signed int32|16 samples summed - signed int32|32 samples summed - signed int32|64 samples summed - signed int32|128 samples summed - signed int32|256 samples summed - signed int32),popup(Not used|unsigned int16 |signed int16|unsigned int32|signed int32|---BurstSample with internal Digital filter---|2 samples averaged - unsigned int16|4 samples averaged - unsigned int16|8 samples averaged - unsigned int16|16 samples averaged - unsigned int16|32 samples averaged - unsigned int16|64 samples averaged - unsigned int16|128 samples averaged - unsigned int16|256 samples averaged - unsigned int16|---|2 samples averaged - signed int16|4 samples averaged - signed int16|8 samples averaged - signed int16|16 samples averaged - signed int16|32 samples averaged - signed int16|64 samples averaged - signed int16|128 samples averaged - signed int16|256 samples averaged - signed int16|---|4 samples summed - unsigned int16|8 samples summed - unsigned int16|16 samples summed - unsigned int16|32 samples summed - unsigned int16|64 samples summed - unsigned int16|128 samples summed - unsigned int16|256 samples summed - unsigned int16|---|2 samples summed - signed int16|4 samples summed - signed int16|8 samples summed - signed int16|16 samples summed - signed int16|32 samples summed - signed int16|64 samples summed - signed int16|128 samples summed - signed int16|256 samples summed - signed int16|---|2 samples averaged - unsigned int32|4 samples averaged - unsigned int32|8 samples averaged - unsigned int32|16 samples averaged - unsigned int32|32 samples averaged - unsigned int32|64 samples averaged - unsigned int32|128 samples averaged - unsigned int32|256 samples averaged - unsigned int32|---|2 samples averaged - signed int32|4 samples averaged - signed int32|8 samples averaged - signed int32|16 samples averaged - signed int32|32 samples averaged - signed int32|64 samples averaged - signed int32|128 samples averaged - signed int32|256 samples averaged - signed int32|---|4 samples summed - unsigned int32|8 samples summed - unsigned int32|16 samples summed - unsigned int32|32 samples summed - unsigned int32|64 samples summed - unsigned int32|128 samples summed - unsigned int32|256 samples summed - unsigned int32|---|2 samples summed - signed int32|4 samples summed - signed int32|8 samples summed - signed int32|16 samples summed - signed int32|32 samples summed - signed int32|64 samples summed - signed int32|128 samples summed - signed int32|256 samples summed - signed int32),popup(Not used|unsigned int16 |signed int16|unsigned int32|signed int32|---BurstSample with internal Digital filter---|2 samples averaged - unsigned int16|4 samples averaged - unsigned int16|8 samples averaged - unsigned int16|16 samples averaged - unsigned int16|32 samples averaged - unsigned int16|64 samples averaged - unsigned int16|128 samples averaged - unsigned int16|256 samples averaged - unsigned int16|---|2 samples averaged - signed int16|4 samples averaged - signed int16|8 samples averaged - signed int16|16 samples averaged - signed int16|32 samples averaged - signed int16|64 samples averaged - signed int16|128 samples averaged - signed int16|256 samples averaged - signed int16|---|4 samples summed - unsigned int16|8 samples summed - unsigned int16|16 samples summed - unsigned int16|32 samples summed - unsigned int16|64 samples summed - unsigned int16|128 samples summed - unsigned int16|256 samples summed - unsigned int16|---|2 samples summed - signed int16|4 samples summed - signed int16|8 samples summed - signed int16|16 samples summed - signed int16|32 samples summed - signed int16|64 samples summed - signed int16|128 samples summed - signed int16|256 samples summed - signed int16|---|2 samples averaged - unsigned int32|4 samples averaged - unsigned int32|8 samples averaged - unsigned int32|16 samples averaged - unsigned int32|32 samples averaged - unsigned int32|64 samples averaged - unsigned int32|128 samples averaged - unsigned int32|256 samples averaged - unsigned int32|---|2 samples averaged - signed int32|4 samples averaged - signed int32|8 samples averaged - signed int32|16 samples averaged - signed int32|32 samples averaged - signed int32|64 samples averaged - signed int32|128 samples averaged - signed int32|256 samples averaged - signed int32|---|4 samples summed - unsigned int32|8 samples summed - unsigned int32|16 samples summed - unsigned int32|32 samples summed - unsigned int32|64 samples summed - unsigned int32|128 samples summed - unsigned int32|256 samples summed - unsigned int32|---|2 samples summed - signed int32|4 samples summed - signed int32|8 samples summed - signed int32|16 samples summed - signed int32|32 samples summed - signed int32|64 samples summed - signed int32|128 samples summed - signed int32|256 samples summed - signed int32),popup(Not used|unsigned int16 |signed int16|unsigned int32|signed int32|---BurstSample with internal Digital filter---|2 samples averaged - unsigned int16|4 samples averaged - unsigned int16|8 samples averaged - unsigned int16|16 samples averaged - unsigned int16|32 samples averaged - unsigned int16|64 samples averaged - unsigned int16|128 samples averaged - unsigned int16|256 samples averaged - unsigned int16|---|2 samples averaged - signed int16|4 samples averaged - signed int16|8 samples averaged - signed int16|16 samples averaged - signed int16|32 samples averaged - signed int16|64 samples averaged - signed int16|128 samples averaged - signed int16|256 samples averaged - signed int16|---|4 samples summed - unsigned int16|8 samples summed - unsigned int16|16 samples summed - unsigned int16|32 samples summed - unsigned int16|64 samples summed - unsigned int16|128 samples summed - unsigned int16|256 samples summed - unsigned int16|---|2 samples summed - signed int16|4 samples summed - signed int16|8 samples summed - signed int16|16 samples summed - signed int16|32 samples summed - signed int16|64 samples summed - signed int16|128 samples summed - signed int16|256 samples summed - signed int16|---|2 samples averaged - unsigned int32|4 samples averaged - unsigned int32|8 samples averaged - unsigned int32|16 samples averaged - unsigned int32|32 samples averaged - unsigned int32|64 samples averaged - unsigned int32|128 samples averaged - unsigned int32|256 samples averaged - unsigned int32|---|2 samples averaged - signed int32|4 samples averaged - signed int32|8 samples averaged - signed int32|16 samples averaged - signed int32|32 samples averaged - signed int32|64 samples averaged - signed int32|128 samples averaged - signed int32|256 samples averaged - signed int32|---|4 samples summed - unsigned int32|8 samples summed - unsigned int32|16 samples summed - unsigned int32|32 samples summed - unsigned int32|64 samples summed - unsigned int32|128 samples summed - unsigned int32|256 samples summed - unsigned int32|---|2 samples summed - signed int32|4 samples summed - signed int32|8 samples summed - signed int32|16 samples summed - signed int32|32 samples summed - signed int32|64 samples summed - signed int32|128 samples summed - signed int32|256 samples summed - signed int32),popup(Not used|unsigned int16 |signed int16|unsigned int32|signed int32|---BurstSample with internal Digital filter---|2 samples averaged - unsigned int16|4 samples averaged - unsigned int16|8 samples averaged - unsigned int16|16 samples averaged - unsigned int16|32 samples averaged - unsigned int16|64 samples averaged - unsigned int16|128 samples averaged - unsigned int16|256 samples averaged - unsigned int16|---|2 samples averaged - signed int16|4 samples averaged - signed int16|8 samples averaged - signed int16|16 samples averaged - signed int16|32 samples averaged - signed int16|64 samples averaged - signed int16|128 samples averaged - signed int16|256 samples averaged - signed int16|---|4 samples summed - unsigned int16|8 samples summed - unsigned int16|16 samples summed - unsigned int16|32 samples summed - unsigned int16|64 samples summed - unsigned int16|128 samples summed - unsigned int16|256 samples summed - unsigned int16|---|2 samples summed - signed int16|4 samples summed - signed int16|8 samples summed - signed int16|16 samples summed - signed int16|32 samples summed - signed int16|64 samples summed - signed int16|128 samples summed - signed int16|256 samples summed - signed int16|---|2 samples averaged - unsigned int32|4 samples averaged - unsigned int32|8 samples averaged - unsigned int32|16 samples averaged - unsigned int32|32 samples averaged - unsigned int32|64 samples averaged - unsigned int32|128 samples averaged - unsigned int32|256 samples averaged - unsigned int32|---|2 samples averaged - signed int32|4 samples averaged - signed int32|8 samples averaged - signed int32|16 samples averaged - signed int32|32 samples averaged - signed int32|64 samples averaged - signed int32|128 samples averaged - signed int32|256 samples averaged - signed int32|---|4 samples summed - unsigned int32|8 samples summed - unsigned int32|16 samples summed - unsigned int32|32 samples summed - unsigned int32|64 samples summed - unsigned int32|128 samples summed - unsigned int32|256 samples summed - unsigned int32|---|2 samples summed - signed int32|4 samples summed - signed int32|8 samples summed - signed int32|16 samples summed - signed int32|32 samples summed - signed int32|64 samples summed - signed int32|128 samples summed - signed int32|256 samples summed - signed int32),popup(Not used|unsigned int16 |signed int16|unsigned int32|signed int32|---BurstSample with internal Digital filter---|2 samples averaged - unsigned int16|4 samples averaged - unsigned int16|8 samples averaged - unsigned int16|16 samples averaged - unsigned int16|32 samples averaged - unsigned int16|64 samples averaged - unsigned int16|128 samples averaged - unsigned int16|256 samples averaged - unsigned int16|---|2 samples averaged - signed int16|4 samples averaged - signed int16|8 samples averaged - signed int16|16 samples averaged - signed int16|32 samples averaged - signed int16|64 samples averaged - signed int16|128 samples averaged - signed int16|256 samples averaged - signed int16|---|4 samples summed - unsigned int16|8 samples summed - unsigned int16|16 samples summed - unsigned int16|32 samples summed - unsigned int16|64 samples summed - unsigned int16|128 samples summed - unsigned int16|256 samples summed - unsigned int16|---|2 samples summed - signed int16|4 samples summed - signed int16|8 samples summed - signed int16|16 samples summed - signed int16|32 samples summed - signed int16|64 samples summed - signed int16|128 samples summed - signed int16|256 samples summed - signed int16|---|2 samples averaged - unsigned int32|4 samples averaged - unsigned int32|8 samples averaged - unsigned int32|16 samples averaged - unsigned int32|32 samples averaged - unsigned int32|64 samples averaged - unsigned int32|128 samples averaged - unsigned int32|256 samples averaged - unsigned int32|---|2 samples averaged - signed int32|4 samples averaged - signed int32|8 samples averaged - signed int32|16 samples averaged - signed int32|32 samples averaged - signed int32|64 samples averaged - signed int32|128 samples averaged - signed int32|256 samples averaged - signed int32|---|4 samples summed - unsigned int32|8 samples summed - unsigned int32|16 samples summed - unsigned int32|32 samples summed - unsigned int32|64 samples summed - unsigned int32|128 samples summed - unsigned int32|256 samples summed - unsigned int32|---|2 samples summed - signed int32|4 samples summed - signed int32|8 samples summed - signed int32|16 samples summed - signed int32|32 samples summed - signed int32|64 samples summed - signed int32|128 samples summed - signed int32|256 samples summed - signed int32),popup(Not used|unsigned int16 |signed int16|unsigned int32|signed int32|---BurstSample with internal Digital filter---|2 samples averaged - unsigned int16|4 samples averaged - unsigned int16|8 samples averaged - unsigned int16|16 samples averaged - unsigned int16|32 samples averaged - unsigned int16|64 samples averaged - unsigned int16|128 samples averaged - unsigned int16|256 samples averaged - unsigned int16|---|2 samples averaged - signed int16|4 samples averaged - signed int16|8 samples averaged - signed int16|16 samples averaged - signed int16|32 samples averaged - signed int16|64 samples averaged - signed int16|128 samples averaged - signed int16|256 samples averaged - signed int16|---|4 samples summed - unsigned int16|8 samples summed - unsigned int16|16 samples summed - unsigned int16|32 samples summed - unsigned int16|64 samples summed - unsigned int16|128 samples summed - unsigned int16|256 samples summed - unsigned int16|---|2 samples summed - signed int16|4 samples summed - signed int16|8 samples summed - signed int16|16 samples summed - signed int16|32 samples summed - signed int16|64 samples summed - signed int16|128 samples summed - signed int16|256 samples summed - signed int16|---|2 samples averaged - unsigned int32|4 samples averaged - unsigned int32|8 samples averaged - unsigned int32|16 samples averaged - unsigned int32|32 samples averaged - unsigned int32|64 samples averaged - unsigned int32|128 samples averaged - unsigned int32|256 samples averaged - unsigned int32|---|2 samples averaged - signed int32|4 samples averaged - signed int32|8 samples averaged - signed int32|16 samples averaged - signed int32|32 samples averaged - signed int32|64 samples averaged - signed int32|128 samples averaged - signed int32|256 samples averaged - signed int32|---|4 samples summed - unsigned int32|8 samples summed - unsigned int32|16 samples summed - unsigned int32|32 samples summed - unsigned int32|64 samples summed - unsigned int32|128 samples summed - unsigned int32|256 samples summed - unsigned int32|---|2 samples summed - signed int32|4 samples summed - signed int32|8 samples summed - signed int32|16 samples summed - signed int32|32 samples summed - signed int32|64 samples summed - signed int32|128 samples summed - signed int32|256 samples summed - signed int32),popup(Not used|unsigned int16 |signed int16|unsigned int32|signed int32|---BurstSample with internal Digital filter---|2 samples averaged - unsigned int16|4 samples averaged - unsigned int16|8 samples averaged - unsigned int16|16 samples averaged - unsigned int16|32 samples averaged - unsigned int16|64 samples averaged - unsigned int16|128 samples averaged - unsigned int16|256 samples averaged - unsigned int16|---|2 samples averaged - signed int16|4 samples averaged - signed int16|8 samples averaged - signed int16|16 samples averaged - signed int16|32 samples averaged - signed int16|64 samples averaged - signed int16|128 samples averaged - signed int16|256 samples averaged - signed int16|---|4 samples summed - unsigned int16|8 samples summed - unsigned int16|16 samples summed - unsigned int16|32 samples summed - unsigned int16|64 samples summed - unsigned int16|128 samples summed - unsigned int16|256 samples summed - unsigned int16|---|2 samples summed - signed int16|4 samples summed - signed int16|8 samples summed - signed int16|16 samples summed - signed int16|32 samples summed - signed int16|64 samples summed - signed int16|128 samples summed - signed int16|256 samples summed - signed int16|---|2 samples averaged - unsigned int32|4 samples averaged - unsigned int32|8 samples averaged - unsigned int32|16 samples averaged - unsigned int32|32 samples averaged - unsigned int32|64 samples averaged - unsigned int32|128 samples averaged - unsigned int32|256 samples averaged - unsigned int32|---|2 samples averaged - signed int32|4 samples averaged - signed int32|8 samples averaged - signed int32|16 samples averaged - signed int32|32 samples averaged - signed int32|64 samples averaged - signed int32|128 samples averaged - signed int32|256 samples averaged - signed int32|---|4 samples summed - unsigned int32|8 samples summed - unsigned int32|16 samples summed - unsigned int32|32 samples summed - unsigned int32|64 samples summed - unsigned int32|128 samples summed - unsigned int32|256 samples summed - unsigned int32|---|2 samples summed - signed int32|4 samples summed - signed int32|8 samples summed - signed int32|16 samples summed - signed int32|32 samples summed - signed int32|64 samples summed - signed int32|128 samples summed - signed int32|256 samples summed - signed int32),popup(Not used|unsigned int16 |signed int16|unsigned int32|signed int32|---BurstSample with internal Digital filter---|2 samples averaged - unsigned int16|4 samples averaged - unsigned int16|8 samples averaged - unsigned int16|16 samples averaged - unsigned int16|32 samples averaged - unsigned int16|64 samples averaged - unsigned int16|128 samples averaged - unsigned int16|256 samples averaged - unsigned int16|---|2 samples averaged - signed int16|4 samples averaged - signed int16|8 samples averaged - signed int16|16 samples averaged - signed int16|32 samples averaged - signed int16|64 samples averaged - signed int16|128 samples averaged - signed int16|256 samples averaged - signed int16|---|4 samples summed - unsigned int16|8 samples summed - unsigned int16|16 samples summed - unsigned int16|32 samples summed - unsigned int16|64 samples summed - unsigned int16|128 samples summed - unsigned int16|256 samples summed - unsigned int16|---|2 samples summed - signed int16|4 samples summed - signed int16|8 samples summed - signed int16|16 samples summed - signed int16|32 samples summed - signed int16|64 samples summed - signed int16|128 samples summed - signed int16|256 samples summed - signed int16|---|2 samples averaged - unsigned int32|4 samples averaged - unsigned int32|8 samples averaged - unsigned int32|16 samples averaged - unsigned int32|32 samples averaged - unsigned int32|64 samples averaged - unsigned int32|128 samples averaged - unsigned int32|256 samples averaged - unsigned int32|---|2 samples averaged - signed int32|4 samples averaged - signed int32|8 samples averaged - signed int32|16 samples averaged - signed int32|32 samples averaged - signed int32|64 samples averaged - signed int32|128 samples averaged - signed int32|256 samples averaged - signed int32|---|4 samples summed - unsigned int32|8 samples summed - unsigned int32|16 samples summed - unsigned int32|32 samples summed - unsigned int32|64 samples summed - unsigned int32|128 samples summed - unsigned int32|256 samples summed - unsigned int32|---|2 samples summed - signed int32|4 samples summed - signed int32|8 samples summed - signed int32|16 samples summed - signed int32|32 samples summed - signed int32|64 samples summed - signed int32|128 samples summed - signed int32|256 samples summed - signed int32),popup(Not used|unsigned int16 |signed int16|unsigned int32|signed int32|---BurstSample with internal Digital filter---|2 samples averaged - unsigned int16|4 samples averaged - unsigned int16|8 samples averaged - unsigned int16|16 samples averaged - unsigned int16|32 samples averaged - unsigned int16|64 samples averaged - unsigned int16|128 samples averaged - unsigned int16|256 samples averaged - unsigned int16|---|2 samples averaged - signed int16|4 samples averaged - signed int16|8 samples averaged - signed int16|16 samples averaged - signed int16|32 samples averaged - signed int16|64 samples averaged - signed int16|128 samples averaged - signed int16|256 samples averaged - signed int16|---|4 samples summed - unsigned int16|8 samples summed - unsigned int16|16 samples summed - unsigned int16|32 samples summed - unsigned int16|64 samples summed - unsigned int16|128 samples summed - unsigned int16|256 samples summed - unsigned int16|---|2 samples summed - signed int16|4 samples summed - signed int16|8 samples summed - signed int16|16 samples summed - signed int16|32 samples summed - signed int16|64 samples summed - signed int16|128 samples summed - signed int16|256 samples summed - signed int16|---|2 samples averaged - unsigned int32|4 samples averaged - unsigned int32|8 samples averaged - unsigned int32|16 samples averaged - unsigned int32|32 samples averaged - unsigned int32|64 samples averaged - unsigned int32|128 samples averaged - unsigned int32|256 samples averaged - unsigned int32|---|2 samples averaged - signed int32|4 samples averaged - signed int32|8 samples averaged - signed int32|16 samples averaged - signed int32|32 samples averaged - signed int32|64 samples averaged - signed int32|128 samples averaged - signed int32|256 samples averaged - signed int32|---|4 samples summed - unsigned int32|8 samples summed - unsigned int32|16 samples summed - unsigned int32|32 samples summed - unsigned int32|64 samples summed - unsigned int32|128 samples summed - unsigned int32|256 samples summed - unsigned int32|---|2 samples summed - signed int32|4 samples summed - signed int32|8 samples summed - signed int32|16 samples summed - signed int32|32 samples summed - signed int32|64 samples summed - signed int32|128 samples summed - signed int32|256 samples summed - signed int32),popup(Not used|unsigned int16 |signed int16|unsigned int32|signed int32|---BurstSample with internal Digital filter---|2 samples averaged - unsigned int16|4 samples averaged - unsigned int16|8 samples averaged - unsigned int16|16 samples averaged - unsigned int16|32 samples averaged - unsigned int16|64 samples averaged - unsigned int16|128 samples averaged - unsigned int16|256 samples averaged - unsigned int16|---|2 samples averaged - signed int16|4 samples averaged - signed int16|8 samples averaged - signed int16|16 samples averaged - signed int16|32 samples averaged - signed int16|64 samples averaged - signed int16|128 samples averaged - signed int16|256 samples averaged - signed int16|---|4 samples summed - unsigned int16|8 samples summed - unsigned int16|16 samples summed - unsigned int16|32 samples summed - unsigned int16|64 samples summed - unsigned int16|128 samples summed - unsigned int16|256 samples summed - unsigned int16|---|2 samples summed - signed int16|4 samples summed - signed int16|8 samples summed - signed int16|16 samples summed - signed int16|32 samples summed - signed int16|64 samples summed - signed int16|128 samples summed - signed int16|256 samples summed - signed int16|---|2 samples averaged - unsigned int32|4 samples averaged - unsigned int32|8 samples averaged - unsigned int32|16 samples averaged - unsigned int32|32 samples averaged - unsigned int32|64 samples averaged - unsigned int32|128 samples averaged - unsigned int32|256 samples averaged - unsigned int32|---|2 samples averaged - signed int32|4 samples averaged - signed int32|8 samples averaged - signed int32|16 samples averaged - signed int32|32 samples averaged - signed int32|64 samples averaged - signed int32|128 samples averaged - signed int32|256 samples averaged - signed int32|---|4 samples summed - unsigned int32|8 samples summed - unsigned int32|16 samples summed - unsigned int32|32 samples summed - unsigned int32|64 samples summed - unsigned int32|128 samples summed - unsigned int32|256 samples summed - unsigned int32|---|2 samples summed - signed int32|4 samples summed - signed int32|8 samples summed - signed int32|16 samples summed - signed int32|32 samples summed - signed int32|64 samples summed - signed int32|128 samples summed - signed int32|256 samples summed - signed int32),popup(Not used|unsigned int16 |signed int16|unsigned int32|signed int32|---BurstSample with internal Digital filter---|2 samples averaged - unsigned int16|4 samples averaged - unsigned int16|8 samples averaged - unsigned int16|16 samples averaged - unsigned int16|32 samples averaged - unsigned int16|64 samples averaged - unsigned int16|128 samples averaged - unsigned int16|256 samples averaged - unsigned int16|---|2 samples averaged - signed int16|4 samples averaged - signed int16|8 samples averaged - signed int16|16 samples averaged - signed int16|32 samples averaged - signed int16|64 samples averaged - signed int16|128 samples averaged - signed int16|256 samples averaged - signed int16|---|4 samples summed - unsigned int16|8 samples summed - unsigned int16|16 samples summed - unsigned int16|32 samples summed - unsigned int16|64 samples summed - unsigned int16|128 samples summed - unsigned int16|256 samples summed - unsigned int16|---|2 samples summed - signed int16|4 samples summed - signed int16|8 samples summed - signed int16|16 samples summed - signed int16|32 samples summed - signed int16|64 samples summed - signed int16|128 samples summed - signed int16|256 samples summed - signed int16|---|2 samples averaged - unsigned int32|4 samples averaged - unsigned int32|8 samples averaged - unsigned int32|16 samples averaged - unsigned int32|32 samples averaged - unsigned int32|64 samples averaged - unsigned int32|128 samples averaged - unsigned int32|256 samples averaged - unsigned int32|---|2 samples averaged - signed int32|4 samples averaged - signed int32|8 samples averaged - signed int32|16 samples averaged - signed int32|32 samples averaged - signed int32|64 samples averaged - signed int32|128 samples averaged - signed int32|256 samples averaged - signed int32|---|4 samples summed - unsigned int32|8 samples summed - unsigned int32|16 samples summed - unsigned int32|32 samples summed - unsigned int32|64 samples summed - unsigned int32|128 samples summed - unsigned int32|256 samples summed - unsigned int32|---|2 samples summed - signed int32|4 samples summed - signed int32|8 samples summed - signed int32|16 samples summed - signed int32|32 samples summed - signed int32|64 samples summed - signed int32|128 samples summed - signed int32|256 samples summed - signed int32),popup(Not used|unsigned int16 |signed int16|unsigned int32|signed int32|---BurstSample with internal Digital filter---|2 samples averaged - unsigned int16|4 samples averaged - unsigned int16|8 samples averaged - unsigned int16|16 samples averaged - unsigned int16|32 samples averaged - unsigned int16|64 samples averaged - unsigned int16|128 samples averaged - unsigned int16|256 samples averaged - unsigned int16|---|2 samples averaged - signed int16|4 samples averaged - signed int16|8 samples averaged - signed int16|16 samples averaged - signed int16|32 samples averaged - signed int16|64 samples averaged - signed int16|128 samples averaged - signed int16|256 samples averaged - signed int16|---|4 samples summed - unsigned int16|8 samples summed - unsigned int16|16 samples summed - unsigned int16|32 samples summed - unsigned int16|64 samples summed - unsigned int16|128 samples summed - unsigned int16|256 samples summed - unsigned int16|---|2 samples summed - signed int16|4 samples summed - signed int16|8 samples summed - signed int16|16 samples summed - signed int16|32 samples summed - signed int16|64 samples summed - signed int16|128 samples summed - signed int16|256 samples summed - signed int16|---|2 samples averaged - unsigned int32|4 samples averaged - unsigned int32|8 samples averaged - unsigned int32|16 samples averaged - unsigned int32|32 samples averaged - unsigned int32|64 samples averaged - unsigned int32|128 samples averaged - unsigned int32|256 samples averaged - unsigned int32|---|2 samples averaged - signed int32|4 samples averaged - signed int32|8 samples averaged - signed int32|16 samples averaged - signed int32|32 samples averaged - signed int32|64 samples averaged - signed int32|128 samples averaged - signed int32|256 samples averaged - signed int32|---|4 samples summed - unsigned int32|8 samples summed - unsigned int32|16 samples summed - unsigned int32|32 samples summed - unsigned int32|64 samples summed - unsigned int32|128 samples summed - unsigned int32|256 samples summed - unsigned int32|---|2 samples summed - signed int32|4 samples summed - signed int32|8 samples summed - signed int32|16 samples summed - signed int32|32 samples summed - signed int32|64 samples summed - signed int32|128 samples summed - signed int32|256 samples summed - signed int32),popup(Not used|unsigned int16 |signed int16|unsigned int32|signed int32|---BurstSample with internal Digital filter---|2 samples averaged - unsigned int16|4 samples averaged - unsigned int16|8 samples averaged - unsigned int16|16 samples averaged - unsigned int16|32 samples averaged - unsigned int16|64 samples averaged - unsigned int16|128 samples averaged - unsigned int16|256 samples averaged - unsigned int16|---|2 samples averaged - signed int16|4 samples averaged - signed int16|8 samples averaged - signed int16|16 samples averaged - signed int16|32 samples averaged - signed int16|64 samples averaged - signed int16|128 samples averaged - signed int16|256 samples averaged - signed int16|---|4 samples summed - unsigned int16|8 samples summed - unsigned int16|16 samples summed - unsigned int16|32 samples summed - unsigned int16|64 samples summed - unsigned int16|128 samples summed - unsigned int16|256 samples summed - unsigned int16|---|2 samples summed - signed int16|4 samples summed - signed int16|8 samples summed - signed int16|16 samples summed - signed int16|32 samples summed - signed int16|64 samples summed - signed int16|128 samples summed - signed int16|256 samples summed - signed int16|---|2 samples averaged - unsigned int32|4 samples averaged - unsigned int32|8 samples averaged - unsigned int32|16 samples averaged - unsigned int32|32 samples averaged - unsigned int32|64 samples averaged - unsigned int32|128 samples averaged - unsigned int32|256 samples averaged - unsigned int32|---|2 samples averaged - signed int32|4 samples averaged - signed int32|8 samples averaged - signed int32|16 samples averaged - signed int32|32 samples averaged - signed int32|64 samples averaged - signed int32|128 samples averaged - signed int32|256 samples averaged - signed int32|---|4 samples summed - unsigned int32|8 samples summed - unsigned int32|16 samples summed - unsigned int32|32 samples summed - unsigned int32|64 samples summed - unsigned int32|128 samples summed - unsigned int32|256 samples summed - unsigned int32|---|2 samples summed - signed int32|4 samples summed - signed int32|8 samples summed - signed int32|16 samples summed - signed int32|32 samples summed - signed int32|64 samples summed - signed int32|128 samples summed - signed int32|256 samples summed - signed int32),popup(Not used|unsigned int16 |signed int16|unsigned int32|signed int32|---BurstSample with internal Digital filter---|2 samples averaged - unsigned int16|4 samples averaged - unsigned int16|8 samples averaged - unsigned int16|16 samples averaged - unsigned int16|32 samples averaged - unsigned int16|64 samples averaged - unsigned int16|128 samples averaged - unsigned int16|256 samples averaged - unsigned int16|---|2 samples averaged - signed int16|4 samples averaged - signed int16|8 samples averaged - signed int16|16 samples averaged - signed int16|32 samples averaged - signed int16|64 samples averaged - signed int16|128 samples averaged - signed int16|256 samples averaged - signed int16|---|4 samples summed - unsigned int16|8 samples summed - unsigned int16|16 samples summed - unsigned int16|32 samples summed - unsigned int16|64 samples summed - unsigned int16|128 samples summed - unsigned int16|256 samples summed - unsigned int16|---|2 samples summed - signed int16|4 samples summed - signed int16|8 samples summed - signed int16|16 samples summed - signed int16|32 samples summed - signed int16|64 samples summed - signed int16|128 samples summed - signed int16|256 samples summed - signed int16|---|2 samples averaged - unsigned int32|4 samples averaged - unsigned int32|8 samples averaged - unsigned int32|16 samples averaged - unsigned int32|32 samples averaged - unsigned int32|64 samples averaged - unsigned int32|128 samples averaged - unsigned int32|256 samples averaged - unsigned int32|---|2 samples averaged - signed int32|4 samples averaged - signed int32|8 samples averaged - signed int32|16 samples averaged - signed int32|32 samples averaged - signed int32|64 samples averaged - signed int32|128 samples averaged - signed int32|256 samples averaged - signed int32|---|4 samples summed - unsigned int32|8 samples summed - unsigned int32|16 samples summed - unsigned int32|32 samples summed - unsigned int32|64 samples summed - unsigned int32|128 samples summed - unsigned int32|256 samples summed - unsigned int32|---|2 samples summed - signed int32|4 samples summed - signed int32|8 samples summed - signed int32|16 samples summed - signed int32|32 samples summed - signed int32|64 samples summed - signed int32|128 samples summed - signed int32|256 samples summed - signed int32),popup(Not used|unsigned int16 |signed int16|unsigned int32|signed int32|---BurstSample with internal Digital filter---|2 samples averaged - unsigned int16|4 samples averaged - unsigned int16|8 samples averaged - unsigned int16|16 samples averaged - unsigned int16|32 samples averaged - unsigned int16|64 samples averaged - unsigned int16|128 samples averaged - unsigned int16|256 samples averaged - unsigned int16|---|2 samples averaged - signed int16|4 samples averaged - signed int16|8 samples averaged - signed int16|16 samples averaged - signed int16|32 samples averaged - signed int16|64 samples averaged - signed int16|128 samples averaged - signed int16|256 samples averaged - signed int16|---|4 samples summed - unsigned int16|8 samples summed - unsigned int16|16 samples summed - unsigned int16|32 samples summed - unsigned int16|64 samples summed - unsigned int16|128 samples summed - unsigned int16|256 samples summed - unsigned int16|---|2 samples summed - signed int16|4 samples summed - signed int16|8 samples summed - signed int16|16 samples summed - signed int16|32 samples summed - signed int16|64 samples summed - signed int16|128 samples summed - signed int16|256 samples summed - signed int16|---|2 samples averaged - unsigned int32|4 samples averaged - unsigned int32|8 samples averaged - unsigned int32|16 samples averaged - unsigned int32|32 samples averaged - unsigned int32|64 samples averaged - unsigned int32|128 samples averaged - unsigned int32|256 samples averaged - unsigned int32|---|2 samples averaged - signed int32|4 samples averaged - signed int32|8 samples averaged - signed int32|16 samples averaged - signed int32|32 samples averaged - signed int32|64 samples averaged - signed int32|128 samples averaged - signed int32|256 samples averaged - signed int32|---|4 samples summed - unsigned int32|8 samples summed - unsigned int32|16 samples summed - unsigned int32|32 samples summed - unsigned int32|64 samples summed - unsigned int32|128 samples summed - unsigned int32|256 samples summed - unsigned int32|---|2 samples summed - signed int32|4 samples summed - signed int32|8 samples summed - signed int32|16 samples summed - signed int32|32 samples summed - signed int32|64 samples summed - signed int32|128 samples summed - signed int32|256 samples summed - signed int32),popup(Not used|unsigned int16 |signed int16|unsigned int32|signed int32|---BurstSample with internal Digital filter---|2 samples averaged - unsigned int16|4 samples averaged - unsigned int16|8 samples averaged - unsigned int16|16 samples averaged - unsigned int16|32 samples averaged - unsigned int16|64 samples averaged - unsigned int16|128 samples averaged - unsigned int16|256 samples averaged - unsigned int16|---|2 samples averaged - signed int16|4 samples averaged - signed int16|8 samples averaged - signed int16|16 samples averaged - signed int16|32 samples averaged - signed int16|64 samples averaged - signed int16|128 samples averaged - signed int16|256 samples averaged - signed int16|---|4 samples summed - unsigned int16|8 samples summed - unsigned int16|16 samples summed - unsigned int16|32 samples summed - unsigned int16|64 samples summed - unsigned int16|128 samples summed - unsigned int16|256 samples summed - unsigned int16|---|2 samples summed - signed int16|4 samples summed - signed int16|8 samples summed - signed int16|16 samples summed - signed int16|32 samples summed - signed int16|64 samples summed - signed int16|128 samples summed - signed int16|256 samples summed - signed int16|---|2 samples averaged - unsigned int32|4 samples averaged - unsigned int32|8 samples averaged - unsigned int32|16 samples averaged - unsigned int32|32 samples averaged - unsigned int32|64 samples averaged - unsigned int32|128 samples averaged - unsigned int32|256 samples averaged - unsigned int32|---|2 samples averaged - signed int32|4 samples averaged - signed int32|8 samples averaged - signed int32|16 samples averaged - signed int32|32 samples averaged - signed int32|64 samples averaged - signed int32|128 samples averaged - signed int32|256 samples averaged - signed int32|---|4 samples summed - unsigned int32|8 samples summed - unsigned int32|16 samples summed - unsigned int32|32 samples summed - unsigned int32|64 samples summed - unsigned int32|128 samples summed - unsigned int32|256 samples summed - unsigned int32|---|2 samples summed - signed int32|4 samples summed - signed int32|8 samples summed - signed int32|16 samples summed - signed int32|32 samples summed - signed int32|64 samples summed - signed int32|128 samples summed - signed int32|256 samples summed - signed int32),popup(Not used|unsigned int16 |signed int16|unsigned int32|signed int32|---BurstSample with internal Digital filter---|2 samples averaged - unsigned int16|4 samples averaged - unsigned int16|8 samples averaged - unsigned int16|16 samples averaged - unsigned int16|32 samples averaged - unsigned int16|64 samples averaged - unsigned int16|128 samples averaged - unsigned int16|256 samples averaged - unsigned int16|---|2 samples averaged - signed int16|4 samples averaged - signed int16|8 samples averaged - signed int16|16 samples averaged - signed int16|32 samples averaged - signed int16|64 samples averaged - signed int16|128 samples averaged - signed int16|256 samples averaged - signed int16|---|4 samples summed - unsigned int16|8 samples summed - unsigned int16|16 samples summed - unsigned int16|32 samples summed - unsigned int16|64 samples summed - unsigned int16|128 samples summed - unsigned int16|256 samples summed - unsigned int16|---|2 samples summed - signed int16|4 samples summed - signed int16|8 samples summed - signed int16|16 samples summed - signed int16|32 samples summed - signed int16|64 samples summed - signed int16|128 samples summed - signed int16|256 samples summed - signed int16|---|2 samples averaged - unsigned int32|4 samples averaged - unsigned int32|8 samples averaged - unsigned int32|16 samples averaged - unsigned int32|32 samples averaged - unsigned int32|64 samples averaged - unsigned int32|128 samples averaged - unsigned int32|256 samples averaged - unsigned int32|---|2 samples averaged - signed int32|4 samples averaged - signed int32|8 samples averaged - signed int32|16 samples averaged - signed int32|32 samples averaged - signed int32|64 samples averaged - signed int32|128 samples averaged - signed int32|256 samples averaged - signed int32|---|4 samples summed - unsigned int32|8 samples summed - unsigned int32|16 samples summed - unsigned int32|32 samples summed - unsigned int32|64 samples summed - unsigned int32|128 samples summed - unsigned int32|256 samples summed - unsigned int32|---|2 samples summed - signed int32|4 samples summed - signed int32|8 samples summed - signed int32|16 samples summed - signed int32|32 samples summed - signed int32|64 samples summed - signed int32|128 samples summed - signed int32|256 samples summed - signed int32),popup(Not used|unsigned int16 |signed int16|unsigned int32|signed int32|---BurstSample with internal Digital filter---|2 samples averaged - unsigned int16|4 samples averaged - unsigned int16|8 samples averaged - unsigned int16|16 samples averaged - unsigned int16|32 samples averaged - unsigned int16|64 samples averaged - unsigned int16|128 samples averaged - unsigned int16|256 samples averaged - unsigned int16|---|2 samples averaged - signed int16|4 samples averaged - signed int16|8 samples averaged - signed int16|16 samples averaged - signed int16|32 samples averaged - signed int16|64 samples averaged - signed int16|128 samples averaged - signed int16|256 samples averaged - signed int16|---|4 samples summed - unsigned int16|8 samples summed - unsigned int16|16 samples summed - unsigned int16|32 samples summed - unsigned int16|64 samples summed - unsigned int16|128 samples summed - unsigned int16|256 samples summed - unsigned int16|---|2 samples summed - signed int16|4 samples summed - signed int16|8 samples summed - signed int16|16 samples summed - signed int16|32 samples summed - signed int16|64 samples summed - signed int16|128 samples summed - signed int16|256 samples summed - signed int16|---|2 samples averaged - unsigned int32|4 samples averaged - unsigned int32|8 samples averaged - unsigned int32|16 samples averaged - unsigned int32|32 samples averaged - unsigned int32|64 samples averaged - unsigned int32|128 samples averaged - unsigned int32|256 samples averaged - unsigned int32|---|2 samples averaged - signed int32|4 samples averaged - signed int32|8 samples averaged - signed int32|16 samples averaged - signed int32|32 samples averaged - signed int32|64 samples averaged - signed int32|128 samples averaged - signed int32|256 samples averaged - signed int32|---|4 samples summed - unsigned int32|8 samples summed - unsigned int32|16 samples summed - unsigned int32|32 samples summed - unsigned int32|64 samples summed - unsigned int32|128 samples summed - unsigned int32|256 samples summed - unsigned int32|---|2 samples summed - signed int32|4 samples summed - signed int32|8 samples summed - signed int32|16 samples summed - signed int32|32 samples summed - signed int32|64 samples summed - signed int32|128 samples summed - signed int32|256 samples summed - signed int32),popup(Not used|unsigned int16 |signed int16|unsigned int32|signed int32|---BurstSample with internal Digital filter---|2 samples averaged - unsigned int16|4 samples averaged - unsigned int16|8 samples averaged - unsigned int16|16 samples averaged - unsigned int16|32 samples averaged - unsigned int16|64 samples averaged - unsigned int16|128 samples averaged - unsigned int16|256 samples averaged - unsigned int16|---|2 samples averaged - signed int16|4 samples averaged - signed int16|8 samples averaged - signed int16|16 samples averaged - signed int16|32 samples averaged - signed int16|64 samples averaged - signed int16|128 samples averaged - signed int16|256 samples averaged - signed int16|---|4 samples summed - unsigned int16|8 samples summed - unsigned int16|16 samples summed - unsigned int16|32 samples summed - unsigned int16|64 samples summed - unsigned int16|128 samples summed - unsigned int16|256 samples summed - unsigned int16|---|2 samples summed - signed int16|4 samples summed - signed int16|8 samples summed - signed int16|16 samples summed - signed int16|32 samples summed - signed int16|64 samples summed - signed int16|128 samples summed - signed int16|256 samples summed - signed int16|---|2 samples averaged - unsigned int32|4 samples averaged - unsigned int32|8 samples averaged - unsigned int32|16 samples averaged - unsigned int32|32 samples averaged - unsigned int32|64 samples averaged - unsigned int32|128 samples averaged - unsigned int32|256 samples averaged - unsigned int32|---|2 samples averaged - signed int32|4 samples averaged - signed int32|8 samples averaged - signed int32|16 samples averaged - signed int32|32 samples averaged - signed int32|64 samples averaged - signed int32|128 samples averaged - signed int32|256 samples averaged - signed int32|---|4 samples summed - unsigned int32|8 samples summed - unsigned int32|16 samples summed - unsigned int32|32 samples summed - unsigned int32|64 samples summed - unsigned int32|128 samples summed - unsigned int32|256 samples summed - unsigned int32|---|2 samples summed - signed int32|4 samples summed - signed int32|8 samples summed - signed int32|16 samples summed - signed int32|32 samples summed - signed int32|64 samples summed - signed int32|128 samples summed - signed int32|256 samples summed - signed int32),popup(Not used|unsigned int16 |signed int16|unsigned int32|signed int32|---BurstSample with internal Digital filter---|2 samples averaged - unsigned int16|4 samples averaged - unsigned int16|8 samples averaged - unsigned int16|16 samples averaged - unsigned int16|32 samples averaged - unsigned int16|64 samples averaged - unsigned int16|128 samples averaged - unsigned int16|256 samples averaged - unsigned int16|---|2 samples averaged - signed int16|4 samples averaged - signed int16|8 samples averaged - signed int16|16 samples averaged - signed int16|32 samples averaged - signed int16|64 samples averaged - signed int16|128 samples averaged - signed int16|256 samples averaged - signed int16|---|4 samples summed - unsigned int16|8 samples summed - unsigned int16|16 samples summed - unsigned int16|32 samples summed - unsigned int16|64 samples summed - unsigned int16|128 samples summed - unsigned int16|256 samples summed - unsigned int16|---|2 samples summed - signed int16|4 samples summed - signed int16|8 samples summed - signed int16|16 samples summed - signed int16|32 samples summed - signed int16|64 samples summed - signed int16|128 samples summed - signed int16|256 samples summed - signed int16|---|2 samples averaged - unsigned int32|4 samples averaged - unsigned int32|8 samples averaged - unsigned int32|16 samples averaged - unsigned int32|32 samples averaged - unsigned int32|64 samples averaged - unsigned int32|128 samples averaged - unsigned int32|256 samples averaged - unsigned int32|---|2 samples averaged - signed int32|4 samples averaged - signed int32|8 samples averaged - signed int32|16 samples averaged - signed int32|32 samples averaged - signed int32|64 samples averaged - signed int32|128 samples averaged - signed int32|256 samples averaged - signed int32|---|4 samples summed - unsigned int32|8 samples summed - unsigned int32|16 samples summed - unsigned int32|32 samples summed - unsigned int32|64 samples summed - unsigned int32|128 samples summed - unsigned int32|256 samples summed - unsigned int32|---|2 samples summed - signed int32|4 samples summed - signed int32|8 samples summed - signed int32|16 samples summed - signed int32|32 samples summed - signed int32|64 samples summed - signed int32|128 samples summed - signed int32|256 samples summed - signed int32),popup(Not used|unsigned int16 |signed int16|unsigned int32|signed int32|---BurstSample with internal Digital filter---|2 samples averaged - unsigned int16|4 samples averaged - unsigned int16|8 samples averaged - unsigned int16|16 samples averaged - unsigned int16|32 samples averaged - unsigned int16|64 samples averaged - unsigned int16|128 samples averaged - unsigned int16|256 samples averaged - unsigned int16|---|2 samples averaged - signed int16|4 samples averaged - signed int16|8 samples averaged - signed int16|16 samples averaged - signed int16|32 samples averaged - signed int16|64 samples averaged - signed int16|128 samples averaged - signed int16|256 samples averaged - signed int16|---|4 samples summed - unsigned int16|8 samples summed - unsigned int16|16 samples summed - unsigned int16|32 samples summed - unsigned int16|64 samples summed - unsigned int16|128 samples summed - unsigned int16|256 samples summed - unsigned int16|---|2 samples summed - signed int16|4 samples summed - signed int16|8 samples summed - signed int16|16 samples summed - signed int16|32 samples summed - signed int16|64 samples summed - signed int16|128 samples summed - signed int16|256 samples summed - signed int16|---|2 samples averaged - unsigned int32|4 samples averaged - unsigned int32|8 samples averaged - unsigned int32|16 samples averaged - unsigned int32|32 samples averaged - unsigned int32|64 samples averaged - unsigned int32|128 samples averaged - unsigned int32|256 samples averaged - unsigned int32|---|2 samples averaged - signed int32|4 samples averaged - signed int32|8 samples averaged - signed int32|16 samples averaged - signed int32|32 samples averaged - signed int32|64 samples averaged - signed int32|128 samples averaged - signed int32|256 samples averaged - signed int32|---|4 samples summed - unsigned int32|8 samples summed - unsigned int32|16 samples summed - unsigned int32|32 samples summed - unsigned int32|64 samples summed - unsigned int32|128 samples summed - unsigned int32|256 samples summed - unsigned int32|---|2 samples summed - signed int32|4 samples summed - signed int32|8 samples summed - signed int32|16 samples summed - signed int32|32 samples summed - signed int32|64 samples summed - signed int32|128 samples summed - signed int32|256 samples summed - signed int32),popup(Not used|unsigned int16 |signed int16|unsigned int32|signed int32|---BurstSample with internal Digital filter---|2 samples averaged - unsigned int16|4 samples averaged - unsigned int16|8 samples averaged - unsigned int16|16 samples averaged - unsigned int16|32 samples averaged - unsigned int16|64 samples averaged - unsigned int16|128 samples averaged - unsigned int16|256 samples averaged - unsigned int16|---|2 samples averaged - signed int16|4 samples averaged - signed int16|8 samples averaged - signed int16|16 samples averaged - signed int16|32 samples averaged - signed int16|64 samples averaged - signed int16|128 samples averaged - signed int16|256 samples averaged - signed int16|---|4 samples summed - unsigned int16|8 samples summed - unsigned int16|16 samples summed - unsigned int16|32 samples summed - unsigned int16|64 samples summed - unsigned int16|128 samples summed - unsigned int16|256 samples summed - unsigned int16|---|2 samples summed - signed int16|4 samples summed - signed int16|8 samples summed - signed int16|16 samples summed - signed int16|32 samples summed - signed int16|64 samples summed - signed int16|128 samples summed - signed int16|256 samples summed - signed int16|---|2 samples averaged - unsigned int32|4 samples averaged - unsigned int32|8 samples averaged - unsigned int32|16 samples averaged - unsigned int32|32 samples averaged - unsigned int32|64 samples averaged - unsigned int32|128 samples averaged - unsigned int32|256 samples averaged - unsigned int32|---|2 samples averaged - signed int32|4 samples averaged - signed int32|8 samples averaged - signed int32|16 samples averaged - signed int32|32 samples averaged - signed int32|64 samples averaged - signed int32|128 samples averaged - signed int32|256 samples averaged - signed int32|---|4 samples summed - unsigned int32|8 samples summed - unsigned int32|16 samples summed - unsigned int32|32 samples summed - unsigned int32|64 samples summed - unsigned int32|128 samples summed - unsigned int32|256 samples summed - unsigned int32|---|2 samples summed - signed int32|4 samples summed - signed int32|8 samples summed - signed int32|16 samples summed - signed int32|32 samples summed - signed int32|64 samples summed - signed int32|128 samples summed - signed int32|256 samples summed - signed int32),popup(Not used|unsigned int16 |signed int16|unsigned int32|signed int32|---BurstSample with internal Digital filter---|2 samples averaged - unsigned int16|4 samples averaged - unsigned int16|8 samples averaged - unsigned int16|16 samples averaged - unsigned int16|32 samples averaged - unsigned int16|64 samples averaged - unsigned int16|128 samples averaged - unsigned int16|256 samples averaged - unsigned int16|---|2 samples averaged - signed int16|4 samples averaged - signed int16|8 samples averaged - signed int16|16 samples averaged - signed int16|32 samples averaged - signed int16|64 samples averaged - signed int16|128 samples averaged - signed int16|256 samples averaged - signed int16|---|4 samples summed - unsigned int16|8 samples summed - unsigned int16|16 samples summed - unsigned int16|32 samples summed - unsigned int16|64 samples summed - unsigned int16|128 samples summed - unsigned int16|256 samples summed - unsigned int16|---|2 samples summed - signed int16|4 samples summed - signed int16|8 samples summed - signed int16|16 samples summed - signed int16|32 samples summed - signed int16|64 samples summed - signed int16|128 samples summed - signed int16|256 samples summed - signed int16|---|2 samples averaged - unsigned int32|4 samples averaged - unsigned int32|8 samples averaged - unsigned int32|16 samples averaged - unsigned int32|32 samples averaged - unsigned int32|64 samples averaged - unsigned int32|128 samples averaged - unsigned int32|256 samples averaged - unsigned int32|---|2 samples averaged - signed int32|4 samples averaged - signed int32|8 samples averaged - signed int32|16 samples averaged - signed int32|32 samples averaged - signed int32|64 samples averaged - signed int32|128 samples averaged - signed int32|256 samples averaged - signed int32|---|4 samples summed - unsigned int32|8 samples summed - unsigned int32|16 samples summed - unsigned int32|32 samples summed - unsigned int32|64 samples summed - unsigned int32|128 samples summed - unsigned int32|256 samples summed - unsigned int32|---|2 samples summed - signed int32|4 samples summed - signed int32|8 samples summed - signed int32|16 samples summed - signed int32|32 samples summed - signed int32|64 samples summed - signed int32|128 samples summed - signed int32|256 samples summed - signed int32),popup(Not used|unsigned int16 |signed int16|unsigned int32|signed int32|---BurstSample with internal Digital filter---|2 samples averaged - unsigned int16|4 samples averaged - unsigned int16|8 samples averaged - unsigned int16|16 samples averaged - unsigned int16|32 samples averaged - unsigned int16|64 samples averaged - unsigned int16|128 samples averaged - unsigned int16|256 samples averaged - unsigned int16|---|2 samples averaged - signed int16|4 samples averaged - signed int16|8 samples averaged - signed int16|16 samples averaged - signed int16|32 samples averaged - signed int16|64 samples averaged - signed int16|128 samples averaged - signed int16|256 samples averaged - signed int16|---|4 samples summed - unsigned int16|8 samples summed - unsigned int16|16 samples summed - unsigned int16|32 samples summed - unsigned int16|64 samples summed - unsigned int16|128 samples summed - unsigned int16|256 samples summed - unsigned int16|---|2 samples summed - signed int16|4 samples summed - signed int16|8 samples summed - signed int16|16 samples summed - signed int16|32 samples summed - signed int16|64 samples summed - signed int16|128 samples summed - signed int16|256 samples summed - signed int16|---|2 samples averaged - unsigned int32|4 samples averaged - unsigned int32|8 samples averaged - unsigned int32|16 samples averaged - unsigned int32|32 samples averaged - unsigned int32|64 samples averaged - unsigned int32|128 samples averaged - unsigned int32|256 samples averaged - unsigned int32|---|2 samples averaged - signed int32|4 samples averaged - signed int32|8 samples averaged - signed int32|16 samples averaged - signed int32|32 samples averaged - signed int32|64 samples averaged - signed int32|128 samples averaged - signed int32|256 samples averaged - signed int32|---|4 samples summed - unsigned int32|8 samples summed - unsigned int32|16 samples summed - unsigned int32|32 samples summed - unsigned int32|64 samples summed - unsigned int32|128 samples summed - unsigned int32|256 samples summed - unsigned int32|---|2 samples summed - signed int32|4 samples summed - signed int32|8 samples summed - signed int32|16 samples summed - signed int32|32 samples summed - signed int32|64 samples summed - signed int32|128 samples summed - signed int32|256 samples summed - signed int32),popup(Not used|unsigned int16 |signed int16|unsigned int32|signed int32),popup(Not used|unsigned int16 |signed int16|unsigned int32|signed int32),popup(Not used|unsigned int16 |signed int16|unsigned int32|signed int32),popup(Not used|unsigned int16 |signed int16|unsigned int32|signed int32),popup(Not used|unsigned int16 |signed int16|unsigned int32|signed int32),popup(Not used|unsigned int16 |signed int16|unsigned int32|signed int32),popup(Not used|unsigned int16 |signed int16|unsigned int32|signed int32),popup(Not used|unsigned int16 |signed int16|unsigned int32|signed int32),popup(Not used|unsigned int16 |signed int16|unsigned int32|signed int32),popup(Not used|unsigned int16 |signed int16|unsigned int32|signed int32),popup(Not used|unsigned int16 |signed int16|unsigned int32|signed int32),popup(Not used|unsigned int16 |signed int16|unsigned int32|signed int32),popup(Not used|unsigned int16 |signed int16|unsigned int32|signed int32),popup(Not used|unsigned int16 |signed int16|unsigned int32|signed int32),popup(Not used|unsigned int16 |signed int16|unsigned int32|signed int32),popup(Not used|unsigned int16 |signed int16|unsigned int32|signed int32),popup(Not used|unsigned int16 |signed int16|unsigned int32|signed int32),popup(Not used|unsigned int16 |signed int16|unsigned int32|signed int32),popup(Not used|unsigned int16 |signed int16|unsigned int32|signed int32),popup(Not used|unsigned int16 |signed int16|unsigned int32|signed int32),popup(Not used|unsigned int16 |signed int16|unsigned int32|signed int32),popup(Not used|unsigned int16 |signed int16|unsigned int32|signed int32),popup(Not used|unsigned int16 |signed int16|unsigned int32|signed int32),popup(Not used|unsigned int16 |signed int16|unsigned int32|signed int32),popup(Not used|unsigned int16 |signed int16|unsigned int32|signed int32),popup(Not used|unsigned int16 |signed int16|unsigned int32|signed int32),popup(Not used|unsigned int16 |signed int16|unsigned int32|signed int32),popup(Not used|unsigned int16 |signed int16|unsigned int32|signed int32),popup(Not used|unsigned int16 |signed int16|unsigned int32|signed int32),popup(Not used|unsigned int16 |signed int16|unsigned int32|signed int32),popup(Not used|unsigned int16 |signed int16|unsigned int32|signed int32),popup(Not used|unsigned int16 |signed int16|unsigned int32|signed int32),popup(Not used|unsigned int16 |unsigned int32),popup(Not used|unsigned int16 |unsigned int32),popup(Not used|unsigned int16 |unsigned int32),popup(Not used|unsigned int16 |unsigned int32)
      mask CallbackString: ||||MCHP_ADC_HighSpeed_SAR_Callback(gcbh,'DialogUpdate');||||||||||||||||MCHP_ADC_HighSpeed_SAR_Callback(gcbh,'DialogUpdate');|||||MCHP_ADC_HighSpeed_SAR_Callback(gcbh,'DialogUpdate');|||||MCHP_ADC_HighSpeed_SAR_Callback(gcbh,'DialogUpdate');|||||MCHP_ADC_HighSpeed_SAR_Callback(gcbh,'DialogUpdate');|||||MCHP_ADC_HighSpeed_SAR_Callback(gcbh,'DialogUpdate');|||||MCHP_ADC_HighSpeed_SAR_Callback(gcbh,'DialogUpdate');|||||MCHP_ADC_HighSpeed_SAR_Callback(gcbh,'DialogUpdate');|||||MCHP_ADC_HighSpeed_SAR_Callback(gcbh,'DialogUpdate');|||||MCHP_ADC_HighSpeed_SAR_Callback(gcbh,'DialogUpdate');|||||MCHP_ADC_HighSpeed_SAR_Callback(gcbh,'DialogUpdate');|||||MCHP_ADC_HighSpeed_SAR_Callback(gcbh,'DialogUpdate');|||||MCHP_ADC_HighSpeed_SAR_Callback(gcbh,'DialogUpdate');|||||MCHP_ADC_HighSpeed_SAR_Callback(gcbh,'DialogUpdate');|||||MCHP_ADC_HighSpeed_SAR_Callback(gcbh,'DialogUpdate');||||||||||||||||||||||||||||||||||||||||||||||||||||||||||||||||||||||||||
      mask TabNameString: ADC main,ADC main,ADC main,ADC main,ADC main,ADC main,ADC main,ADC main,ADC main,ADC main,ADC main,ADC main,ADC main,ADC main,ADC main,ADC main,ADC main,ADC main,ADC main,ADC main,ADC0,ADC0,ADC0,ADC0,ADC0,ADC0,ADC0,ADC0,ADC0,ADC0,ADC1,ADC1,ADC1,ADC1,ADC1,ADC1,ADC1,ADC1,ADC1,ADC1,ADC2,ADC2,ADC2,ADC2,ADC2,ADC2,ADC2,ADC2,ADC2,ADC2,ADC3,ADC3,ADC3,ADC3,ADC3,ADC3,ADC3,ADC3,ADC3,ADC3,ADC4,ADC4,ADC4,ADC4,ADC4,ADC4,ADC4,ADC4,ADC4,ADC4,ADC5,ADC5,ADC5,ADC5,ADC5,ADC5,ADC5,ADC5,ADC5,ADC5,ADC6,ADC6,ADC6,ADC6,ADC6,ADC6,ADC6,ADC6,ADC6,ADC6,ADC7-Class2,ADC7-Class2,ADC7-Class2,ADC7-Class2,ADC7-Class2,ADC7-Class2,ADC7-Class2,ADC7-Class2,ADC7-Class2,ADC7-Class2,ADC7-Class2,ADC7-Class2,ADC7-Class2,ADC7-Class2,ADC7-Class2,ADC7-Class2,ADC7-Class2,ADC7-Class2,ADC7-Class2,ADC7-Class2,ADC7-Class2,ADC7-Class2,ADC7-Class2,ADC7-Class2,ADC7-Class2,ADC7-Class2,ADC7-Class2,ADC7-Class2,ADC7-Class2,ADC7-Class2,ADC7-Class2,ADC7-Class2,ADC7-Class2,ADC7-Class2,ADC7-Class3,ADC7-Class3,ADC7-Class3,ADC7-Class3,ADC7-Class3,ADC7-Class3,ADC7-Class3,ADC7-Class3,ADC7-Class3,ADC7-Class3,ADC7-Class3,ADC7-Class3,ADC7-Class3,ADC7-Class3,ADC7-Class3,ADC7-Class3,ADC7-Class3,ADC7-Class3,ADC7-Class3,ADC7-Class3,ADC7-Class3,ADC7-Class3,ADC7-Class3,ADC7-Class3,ADC7-Class3,ADC7-Class3,ADC7-Class3,ADC7-Class3,ADC7-Class3,ADC7-Class3,ADC7-Class3,ADC7-Class3,ADC7-Class3,ADC7-Class3,ADC7-Class3,ADC7-Class3
      mask Display:
      | fprintf('ADC\nPIC32 EF');
      | port_label('output',1,'AN0');
      | port_label('output',2,'AN1');
  ADC SAMx5 SAMC2x : S-Function  InitFcn=MCHP_ADC_SAME5x_Callback(gcb,'InitFcn');  FunctionName=MCHP_ADC_SAME5x  Parameters=MCHP_ADC_SAME5x_Callback(gcbh,'S_INPUT'),MCHP_ADC_SAME5x_Callback(gcbh,'S_OUTPUT'),MCHP_ADC_SAME5x_Callback(gcbh,'S_INPUT_Size'),MCHP_ADC_SAME5x_Callback(gcbh,'S_OUTPUT_Size'),MCHP_ADC_SAME5x_Callback(gcbh,'S_ListCustomDatatype'),SampleTime,0  EnableBusSupport=off  mask(ADC for SAMD5/E5 & SAMC2x){ADCREF=ADC 0 and ADC 1 (slave), VREF_seq0=Dynamic Options, VREF_seq0_TXT=PA03 / VREFA / Pin[10], info=0, SampleTime=.001, MCHP_PORT={ADC0_AIN1}{ADC0_AIN6}15:2:P6;, MCHP_MASTERLINK=SAME5x_PIM_MCLV2_ADC_R2014b/Microchip Master, MCHP_CRC=, TrigSource_seq0=Dynamic Options, TrigSource_seq0_TXT=, ADC0_seq0=Dynamic Options, ADC0_seq0_TXT=PA06 / AIN6 / Pin[23], ADC1_seq0=Dynamic Options, ADC1_seq0_TXT=PB06 / AIN8 / Pin[17], ADC0_seq0_1=Dynamic Options, ADC0_seq0_1_TXT=Not Used, ADC1_seq0_1=Dynamic Options, ADC1_seq0_1_TXT=Not Used, ADC0_seq0_2=Dynamic Options, ADC0_seq0_2_TXT=Not Used, ADC1_seq0_2=Dynamic Options, ADC1_seq0_2_TXT=Not Used, ADC0_seq0_3=Dynamic Options, ADC0_seq0_3_TXT=Not Used, ADC1_seq0_3=Dynamic Options, ADC1_seq0_3_TXT=Not Used, ADC0_seq0_4=Dynamic Options, ADC0_seq0_4_TXT=Not Used, ADC1_seq0_4=Dynamic Options, ADC1_seq0_4_TXT=Not Used, ADC0_seq0_5=Dynamic Options, ADC0_seq0_5_TXT=Not Used, ADC1_seq0_5=Dynamic Options, ADC1_seq0_5_TXT=Not Used, Resolution_seq0=12 bits, SampleTime_seq0_s=1e-6, TrigTimeStep_seq0=off, info_seq0=0, TrigSource_seq1=Dynamic Options, TrigSource_seq1_TXT=, ADC0_seq1=Dynamic Options, ADC0_seq1_TXT=Not Used, ADC1_seq1=Dynamic Options, ADC1_seq1_TXT=Not Used, ADC0_seq1_1=Dynamic Options, ADC0_seq1_1_TXT=Not Used, ADC1_seq1_1=Dynamic Options, ADC1_seq1_1_TXT=Not Used, ADC0_seq1_2=Dynamic Options, ADC0_seq1_2_TXT=Not Used, ADC1_seq1_2=Dynamic Options, ADC1_seq1_2_TXT=Not Used, ADC0_seq1_3=Dynamic Options, ADC0_seq1_3_TXT=Not Used, ADC1_seq1_3=Dynamic Options, ADC1_seq1_3_TXT=Not Used, ADC0_seq1_4=Dynamic Options, ADC0_seq1_4_TXT=Not Used, ADC1_seq1_4=Dynamic Options, ADC1_seq1_4_TXT=Not Used, ADC0_seq1_5=Dynamic Options, ADC0_seq1_5_TXT=Not Used, ADC1_seq1_5=Dynamic Options, ADC1_seq1_5_TXT=Not Used, Resolution_seq1=12 bits, SampleTime_seq1_s=1e-6, TrigTimeStep_seq1=off, info_seq1=0, TrigSource_seq2=Dynamic Options, TrigSource_seq2_TXT=, ADC0_seq2=Dynamic Options, ADC0_seq2_TXT=Not Used, ADC1_seq2=Dynamic Options, ADC1_seq2_TXT=Not Used, ADC0_seq2_1=Dynamic Options, ADC0_seq2_1_TXT=Not Used, ADC1_seq2_1=Dynamic Options, ADC1_seq2_1_TXT=Not Used, ADC0_seq2_2=Dynamic Options, ADC0_seq2_2_TXT=Not Used, ADC1_seq2_2=Dynamic Options, ADC1_seq2_2_TXT=Not Used, ADC0_seq2_3=Dynamic Options, ADC0_seq2_3_TXT=Not Used, ADC1_seq2_3=Dynamic Options, ADC1_seq2_3_TXT=Not Used, ADC0_seq2_4=Dynamic Options, ADC0_seq2_4_TXT=Not Used, ADC1_seq2_4=Dynamic Options, ADC1_seq2_4_TXT=Not Used, ADC0_seq2_5=Dynamic Options, ADC0_seq2_5_TXT=Not Used, ADC1_seq2_5=Dynamic Options, ADC1_seq2_5_TXT=Not Used, Resolution_seq2=12 bits, SampleTime_seq2_s=1e-6, TrigTimeStep_seq2=off, info_seq2=0, TrigSource_seq3=Dynamic Options, TrigSource_seq3_TXT=, ADC0_seq3=Dynamic Options, ADC0_seq3_TXT=Not Used, ADC1_seq3=Dynamic Options, ADC1_seq3_TXT=Not Used, ADC0_seq3_1=Dynamic Options, ADC0_seq3_1_TXT=Not Used, ADC1_seq3_1=Dynamic Options, ADC1_seq3_1_TXT=Not Used, ADC0_seq3_2=Dynamic Options, ADC0_seq3_2_TXT=Not Used, ADC1_seq3_2=Dynamic Options, ADC1_seq3_2_TXT=Not Used, ADC0_seq3_3=Dynamic Options, ADC0_seq3_3_TXT=Not Used, ADC1_seq3_3=Dynamic Options, ADC1_seq3_3_TXT=Not Used, ADC0_seq3_4=Dynamic Options, ADC0_seq3_4_TXT=Not Used, ADC1_seq3_4=Dynamic Options, ADC1_seq3_4_TXT=Not Used, ADC0_seq3_5=Dynamic Options, ADC0_seq3_5_TXT=Not Used, ADC1_seq3_5=Dynamic Options, ADC1_seq3_5_TXT=Not Used, Resolution_seq3=12 bits, SampleTime_seq3_s=1e-6, TrigTimeStep_seq3=off, info_seq3=0, TrigSource_seq4=Dynamic Options, TrigSource_seq4_TXT=, ADC0_seq4=Dynamic Options, ADC0_seq4_TXT=Not Used, ADC1_seq4=Dynamic Options, ADC1_seq4_TXT=Not Used, ADC0_seq4_1=Dynamic Options, ADC0_seq4_1_TXT=Not Used, ADC1_seq4_1=Dynamic Options, ADC1_seq4_1_TXT=Not Used, ADC0_seq4_2=Dynamic Options, ADC0_seq4_2_TXT=Not Used, ADC1_seq4_2=Dynamic Options, ADC1_seq4_2_TXT=Not Used, ADC0_seq4_3=Dynamic Options, ADC0_seq4_3_TXT=Not Used, ADC1_seq4_3=Dynamic Options, ADC1_seq4_3_TXT=Not Used, ADC0_seq4_4=Dynamic Options, ADC0_seq4_4_TXT=Not Used, ADC1_seq4_4=Dynamic Options, ADC1_seq4_4_TXT=Not Used, ADC0_seq4_5=Dynamic Options, ADC0_seq4_5_TXT=Not Used, ADC1_seq4_5=Dynamic Options, ADC1_seq4_5_TXT=Not Used, Resolution_seq4=12 bits, SampleTime_seq4_s=1e-6, TrigTimeStep_seq4=off, info_seq4=0, TrigSource_seq5=Dynamic Options, TrigSource_seq5_TXT=, ADC0_seq5=Dynamic Options, ADC0_seq5_TXT=Not Used, ADC1_seq5=Dynamic Options, ADC1_seq5_TXT=Not Used, ADC0_seq5_1=Dynamic Options, ADC0_seq5_1_TXT=Not Used, ADC1_seq5_1=Dynamic Options, ADC1_seq5_1_TXT=Not Used, ADC0_seq5_2=Dynamic Options, ADC0_seq5_2_TXT=Not Used, ADC1_seq5_2=Dynamic Options, ADC1_seq5_2_TXT=Not Used, ADC0_seq5_3=Dynamic Options, ADC0_seq5_3_TXT=Not Used, ADC1_seq5_3=Dynamic Options, ADC1_seq5_3_TXT=Not Used, ADC0_seq5_4=Dynamic Options, ADC0_seq5_4_TXT=Not Used, ADC1_seq5_4=Dynamic Options, ADC1_seq5_4_TXT=Not Used, ADC0_seq5_5=Dynamic Options, ADC0_seq5_5_TXT=Not Used, ADC1_seq5_5=Dynamic Options, ADC1_seq5_5_TXT=Not Used, Resolution_seq5=12 bits, SampleTime_seq5_s=1e-6, TrigTimeStep_seq5=off, info_seq5=0}
      mask prompts: ADCREF "ADC peripheral"; VREF_seq0 "VREF_sequence0"; VREF_seq0_TXT "VREF_sequence0"; SampleTime "Block Sample Time"; TrigSource_seq0 "Trigger starting seq 0"; TrigSource_seq0_TXT "Trigger starting seq 0 TXT"; ADC0_seq0 "ADC0 Seq0.0"; ADC0_seq0_TXT "ADC0 Seq0.0"; ADC1_seq0 "ADC1 Seq0.0"; ADC1_seq0_TXT "ADC1 Seq0.0"; ADC0_seq0_1 "ADC0 Seq0.1"; ADC0_seq0_1_TXT "ADC0 Seq0.1"; ADC1_seq0_1 "ADC1 Seq0.1"; ADC1_seq0_1_TXT "ADC1 Seq0.1"; ADC0_seq0_2 "ADC0 Seq0.2"; ADC0_seq0_2_TXT "ADC0 Seq0.2"; ADC1_seq0_2 "ADC1 Seq0.2"; ADC1_seq0_2_TXT "ADC1 Seq0.2"; ADC0_seq0_3 "ADC0 Seq0.3"; ADC0_seq0_3_TXT "ADC0 Seq0.3"; ADC1_seq0_3 "ADC1 Seq0.3"; ADC1_seq0_3_TXT "ADC1 Seq0.3"; ADC0_seq0_4 "ADC0 Seq0.4"; ADC0_seq0_4_TXT "ADC0 Seq0.4"; ADC1_seq0_4 "ADC1 Seq0.4"; ADC1_seq0_4_TXT "ADC1 Seq0.4"; ADC0_seq0_5 "ADC0 Seq0.5"; ADC0_seq0_5_TXT "ADC0 Seq0.5"; ADC1_seq0_5 "ADC1 Seq0.5"; ADC1_seq0_5_TXT "ADC1 Seq0.5"; Resolution_seq0 "Resolution"; SampleTime_seq0_s "ADC Sampling Time"; TrigTimeStep_seq0 "End of seq conversion trig time step"; info_seq0 "seq0 info:"; TrigSource_seq1 "Trigger starting seq 1"; TrigSource_seq1_TXT "Trigger starting seq 1 TXT"; ADC0_seq1 "ADC0 Seq1"; ADC0_seq1_TXT "ADC0 Seq1"; ADC1_seq1 "ADC1 Seq1"; ADC1_seq1_TXT "ADC1 Seq1"; ADC0_seq1_1 "ADC0 Seq1.1"; ADC0_seq1_1_TXT "ADC0 Seq1.1"; ADC1_seq1_1 "ADC1 Seq1.1"; ADC1_seq1_1_TXT "ADC1 Seq1.1"; ADC0_seq1_2 "ADC0 Seq1.2"; ADC0_seq1_2_TXT "ADC0 Seq1.2"; ADC1_seq1_2 "ADC1 Seq1.2"; ADC1_seq1_2_TXT "ADC1 Seq1.2"; ADC0_seq1_3 "ADC0 Seq1.3"; ADC0_seq1_3_TXT "ADC0 Seq1.3"; ADC1_seq1_3 "ADC1 Seq1.3"; ADC1_seq1_3_TXT "ADC1 Seq1.3"; ADC0_seq1_4 "ADC0 Seq1.4"; ADC0_seq1_4_TXT "ADC0 Seq1.4"; ADC1_seq1_4 "ADC1 Seq1.4"; ADC1_seq1_4_TXT "ADC1 Seq1.4"; ADC0_seq1_5 "ADC0 Seq1.5"; ADC0_seq1_5_TXT "ADC0 Seq1.5"; ADC1_seq1_5 "ADC1 Seq1.5"; ADC1_seq1_5_TXT "ADC1 Seq1.5"; Resolution_seq1 "Resolution"; SampleTime_seq1_s "ADC Sampling Time"; TrigTimeStep_seq1 "End of seq conversion trig time step"; info_seq1 "seq1 info:"; TrigSource_seq2 "Trigger starting seq 2"; TrigSource_seq2_TXT "Trigger starting seq 2 TXT"; ADC0_seq2 "ADC0 Seq2"; ADC0_seq2_TXT "ADC0 Seq2"; ADC1_seq2 "ADC1 Seq2"; ADC1_seq2_TXT "ADC1 Seq2"; ADC0_seq2_1 "ADC0 Seq2.1"; ADC0_seq2_1_TXT "ADC0 Seq2.1"; ADC1_seq2_1 "ADC1 Seq2.1"; ADC1_seq2_1_TXT "ADC1 Seq2.1"; ADC0_seq2_2 "ADC0 Seq2.2"; ADC0_seq2_2_TXT "ADC0 Seq2.2"; ADC1_seq2_2 "ADC1 Seq2.2"; ADC1_seq2_2_TXT "ADC1 Seq2.2"; ADC0_seq2_3 "ADC0 Seq2.3"; ADC0_seq2_3_TXT "ADC0 Seq2.3"; ADC1_seq2_3 "ADC1 Seq2.3"; ADC1_seq2_3_TXT "ADC1 Seq2.3"; ADC0_seq2_4 "ADC0 Seq2.4"; ADC0_seq2_4_TXT "ADC0 Seq2.4"; ADC1_seq2_4 "ADC1 Seq2.4"; ADC1_seq2_4_TXT "ADC1 Seq2.4"; ADC0_seq2_5 "ADC0 Seq2.5"; ADC0_seq2_5_TXT "ADC0 Seq2.5"; ADC1_seq2_5 "ADC1 Seq2.5"; ADC1_seq2_5_TXT "ADC1 Seq2.5"; Resolution_seq2 "Resolution"; SampleTime_seq2_s "ADC Sampling Time"; TrigTimeStep_seq2 "End of seq conversion trig time step"; info_seq2 "seq2 info:"; TrigSource_seq3 "Trigger starting seq 3"; TrigSource_seq3_TXT "Trigger starting seq 3 TXT"; ADC0_seq3 "ADC0 Seq3"; ADC0_seq3_TXT "ADC0 Seq3"; ADC1_seq3 "ADC1 Seq3"; ADC1_seq3_TXT "ADC1 Seq3"; ADC0_seq3_1 "ADC0 Seq3.1"; ADC0_seq3_1_TXT "ADC0 Seq3.1"; ADC1_seq3_1 "ADC1 Seq3.1"; ADC1_seq3_1_TXT "ADC1 Seq3.1"; ADC0_seq3_2 "ADC0 Seq3.2"; ADC0_seq3_2_TXT "ADC0 Seq3.2"; ADC1_seq3_2 "ADC1 Seq3.2"; ADC1_seq3_2_TXT "ADC1 Seq3.2"; ADC0_seq3_3 "ADC0 Seq3.3"; ADC0_seq3_3_TXT "ADC0 Seq3.3"; ADC1_seq3_3 "ADC1 Seq3.3"; ADC1_seq3_3_TXT "ADC1 Seq3.3"; ADC0_seq3_4 "ADC0 Seq3.4"; ADC0_seq3_4_TXT "ADC0 Seq3.4"; ADC1_seq3_4 "ADC1 Seq3.4"; ADC1_seq3_4_TXT "ADC1 Seq3.4"; ADC0_seq3_5 "ADC0 Seq3.5"; ADC0_seq3_5_TXT "ADC0 Seq3.5"; ADC1_seq3_5 "ADC1 Seq3.5"; ADC1_seq3_5_TXT "ADC1 Seq3.5"; Resolution_seq3 "Resolution"; SampleTime_seq3_s "ADC Sampling Time"; TrigTimeStep_seq3 "End of seq conversion trig time step"; info_seq3 "seq3 info:"; TrigSource_seq4 "Trigger starting Seq 4"; TrigSource_seq4_TXT "Trigger starting seq 4 TXT"; ADC0_seq4 "ADC0 Seq4"; ADC0_seq4_TXT "ADC0 Seq4"; ADC1_seq4 "ADC1 Seq4"; ADC1_seq4_TXT "ADC1 Seq4"; ADC0_seq4_1 "ADC0 Seq4.1"; ADC0_seq4_1_TXT "ADC0 Seq4.1"; ADC1_seq4_1 "ADC1 Seq4.1"; ADC1_seq4_1_TXT "ADC1 Seq4.1"; ADC0_seq4_2 "ADC0 Seq4.2"; ADC0_seq4_2_TXT "ADC0 Seq4.2"; ADC1_seq4_2 "ADC1 Seq4.2"; ADC1_seq4_2_TXT "ADC1 Seq4.2"; ADC0_seq4_3 "ADC0 Seq4.3"; ADC0_seq4_3_TXT "ADC0 Seq4.3"; ADC1_seq4_3 "ADC1 Seq4.3"; ADC1_seq4_3_TXT "ADC1 Seq4.3"; ADC0_seq4_4 "ADC0 Seq4.4"; ADC0_seq4_4_TXT "ADC0 Seq4.4"; ADC1_seq4_4 "ADC1 Seq4.4"; ADC1_seq4_4_TXT "ADC1 Seq4.4"; ADC0_seq4_5 "ADC0 Seq4.5"; ADC0_seq4_5_TXT "ADC0 Seq4.5"; ADC1_seq4_5 "ADC1 Seq4.5"; ADC1_seq4_5_TXT "ADC1 Seq4.5"; Resolution_seq4 "Resolution"; SampleTime_seq4_s "ADC Sampling Time"; TrigTimeStep_seq4 "End of seq conversion trig time step"; info_seq4 "seq4 info:"; TrigSource_seq5 "Trigger starting seq 5"; TrigSource_seq5_TXT "Trigger starting seq 5"; ADC0_seq5 "ADC0 Seq5"; ADC0_seq5_TXT "ADC0 Seq5"; ADC1_seq5 "ADC1 Seq5"; ADC1_seq5_TXT "ADC1 Seq5"; ADC0_seq5_1 "ADC0 Seq5.1"; ADC0_seq5_1_TXT "ADC0 Seq5.1"; ADC1_seq5_1 "ADC1 Seq5.1"; ADC1_seq5_1_TXT "ADC1 Seq5.1"; ADC0_seq5_2 "ADC0 Seq5.2"; ADC0_seq5_2_TXT "ADC0 Seq5.2"; ADC1_seq5_2 "ADC1 Seq5.2"; ADC1_seq5_2_TXT "ADC1 Seq5.2"; ADC0_seq5_3 "ADC0 Seq5.3"; ADC0_seq5_3_TXT "ADC0 Seq5.3"; ADC1_seq5_3 "ADC1 Seq5.3"; ADC1_seq5_3_TXT "ADC1 Seq5.3"; ADC0_seq5_4 "ADC0 Seq5.4"; ADC0_seq5_4_TXT "ADC0 Seq5.4"; ADC1_seq5_4 "ADC1 Seq5.4"; ADC1_seq5_4_TXT "ADC1 Seq5.4"; ADC0_seq5_5 "ADC0 Seq5.5"; ADC0_seq5_5_TXT "ADC0 Seq5.5"; ADC1_seq5_5 "ADC1 Seq5.5"; ADC1_seq5_5_TXT "ADC1 Seq5.5"; Resolution_seq5 "Resolution"; SampleTime_seq5_s "ADC Sampling Time"; TrigTimeStep_seq5 "End of seq conversion trig time step"; info_seq5 "seq5 info:"
      mask help:
      | Config ADC, ADC0/ADC1. Conversion are done in background.
      | Sequence execute sequentially. A defined trig starts the sequence. End of Sequence can trig the time step.
      | Multiple conversion of one input pin (same ADC) are mapped on one block output.
      | Most recent converted valus is available at block output. All outputs might be refreshed at each time step depending on seq/trig settings.
      mask init:
      | MCHP_ADC_SAME5x_Callback(gcbh,'INITIALISATION');
      settings: CopyFcn=MCHP_Fun.BlockUpdate(gcbh);  DeleteFcn=MCHP_ADC_SAME5x_Callback(gcbh,'DeleteFcn');  PreSaveFcn=MCHP_Fun.PreSaveFcn_DynamicOptions(gcbh);  OpenFcn=MCHP_ADC_SAME5x_Callback(gcb,'OPEN');
      mask StyleString: popup(ADC 0|ADC 1|ADC 0 and ADC 1 (slave)),popup(Dynamic Options),edit,edit,edit,edit,edit,edit,popup(Dynamic Options),edit,popup(Dynamic Options),edit,popup(Dynamic Options),edit,popup(Dynamic Options),edit,popup(Dynamic Options),edit,popup(Dynamic Options),edit,popup(Dynamic Options),edit,popup(Dynamic Options),edit,popup(Dynamic Options),edit,popup(Dynamic Options),edit,popup(Dynamic Options),edit,popup(Dynamic Options),edit,popup(Dynamic Options),edit,popup(12 bits|10 bits|8 bits),edit,checkbox,edit,popup(Dynamic Options),edit,popup(Dynamic Options),edit,popup(Dynamic Options),edit,popup(Dynamic Options),edit,popup(Dynamic Options),edit,popup(Dynamic Options),edit,popup(Dynamic Options),edit,popup(Dynamic Options),edit,popup(Dynamic Options),edit,popup(Dynamic Options),edit,popup(Dynamic Options),edit,popup(Dynamic Options),edit,popup(Dynamic Options),edit,popup(12 bits|10 bits|8 bits),edit,checkbox,edit,popup(Dynamic Options),edit,popup(Dynamic Options),edit,popup(Dynamic Options),edit,popup(Dynamic Options),edit,popup(Dynamic Options),edit,popup(Dynamic Options),edit,popup(Dynamic Options),edit,popup(Dynamic Options),edit,popup(Dynamic Options),edit,popup(Dynamic Options),edit,popup(Dynamic Options),edit,popup(Dynamic Options),edit,popup(Dynamic Options),edit,popup(12 bits|10 bits|8 bits),edit,checkbox,edit,popup(Dynamic Options),edit,popup(Dynamic Options),edit,popup(Dynamic Options),edit,popup(Dynamic Options),edit,popup(Dynamic Options),edit,popup(Dynamic Options),edit,popup(Dynamic Options),edit,popup(Dynamic Options),edit,popup(Dynamic Options),edit,popup(Dynamic Options),edit,popup(Dynamic Options),edit,popup(Dynamic Options),edit,popup(Dynamic Options),edit,popup(12 bits|10 bits|8 bits),edit,checkbox,edit,popup(Dynamic Options),edit,popup(Dynamic Options),edit,popup(Dynamic Options),edit,popup(Dynamic Options),edit,popup(Dynamic Options),edit,popup(Dynamic Options),edit,popup(Dynamic Options),edit,popup(Dynamic Options),edit,popup(Dynamic Options),edit,popup(Dynamic Options),edit,popup(Dynamic Options),edit,popup(Dynamic Options),edit,popup(Dynamic Options),edit,popup(12 bits|10 bits|8 bits),edit,checkbox,edit,popup(Dynamic Options),edit,popup(Dynamic Options),edit,popup(Dynamic Options),edit,popup(Dynamic Options),edit,popup(Dynamic Options),edit,popup(Dynamic Options),edit,popup(Dynamic Options),edit,popup(Dynamic Options),edit,popup(Dynamic Options),edit,popup(Dynamic Options),edit,popup(Dynamic Options),edit,popup(Dynamic Options),edit,popup(Dynamic Options),edit,popup(12 bits|10 bits|8 bits),edit,checkbox,edit
      mask CallbackString: MCHP_ADC_SAME5x_Callback(gcbh,'UpdateGUI');||||||||||MCHP_ADC_SAME5x_Callback(gcbh,'UpdateGUI');||MCHP_ADC_SAME5x_Callback(gcbh,'UpdateGUI');||MCHP_ADC_SAME5x_Callback(gcbh,'UpdateGUI');||MCHP_ADC_SAME5x_Callback(gcbh,'UpdateGUI');||MCHP_ADC_SAME5x_Callback(gcbh,'UpdateGUI');||MCHP_ADC_SAME5x_Callback(gcbh,'UpdateGUI');||MCHP_ADC_SAME5x_Callback(gcbh,'UpdateGUI');||MCHP_ADC_SAME5x_Callback(gcbh,'UpdateGUI');||MCHP_ADC_SAME5x_Callback(gcbh,'UpdateGUI');||MCHP_ADC_SAME5x_Callback(gcbh,'UpdateGUI');||MCHP_ADC_SAME5x_Callback(gcbh,'UpdateGUI');||MCHP_ADC_SAME5x_Callback(gcbh,'UpdateGUI');||||||||MCHP_ADC_SAME5x_Callback(gcbh,'UpdateGUI');||MCHP_ADC_SAME5x_Callback(gcbh,'UpdateGUI');||MCHP_ADC_SAME5x_Callback(gcbh,'UpdateGUI');||MCHP_ADC_SAME5x_Callback(gcbh,'UpdateGUI');||MCHP_ADC_SAME5x_Callback(gcbh,'UpdateGUI');||MCHP_ADC_SAME5x_Callback(gcbh,'UpdateGUI');||MCHP_ADC_SAME5x_Callback(gcbh,'UpdateGUI');||MCHP_ADC_SAME5x_Callback(gcbh,'UpdateGUI');||MCHP_ADC_SAME5x_Callback(gcbh,'UpdateGUI');||MCHP_ADC_SAME5x_Callback(gcbh,'UpdateGUI');||MCHP_ADC_SAME5x_Callback(gcbh,'UpdateGUI');||MCHP_ADC_SAME5x_Callback(gcbh,'UpdateGUI');||||||||MCHP_ADC_SAME5x_Callback(gcbh,'UpdateGUI');||MCHP_ADC_SAME5x_Callback(gcbh,'UpdateGUI');||MCHP_ADC_SAME5x_Callback(gcbh,'UpdateGUI');||MCHP_ADC_SAME5x_Callback(gcbh,'UpdateGUI');||MCHP_ADC_SAME5x_Callback(gcbh,'UpdateGUI');||MCHP_ADC_SAME5x_Callback(gcbh,'UpdateGUI');||MCHP_ADC_SAME5x_Callback(gcbh,'UpdateGUI');||MCHP_ADC_SAME5x_Callback(gcbh,'UpdateGUI');||MCHP_ADC_SAME5x_Callback(gcbh,'UpdateGUI');||MCHP_ADC_SAME5x_Callback(gcbh,'UpdateGUI');||MCHP_ADC_SAME5x_Callback(gcbh,'UpdateGUI');||MCHP_ADC_SAME5x_Callback(gcbh,'UpdateGUI');||||||||MCHP_ADC_SAME5x_Callback(gcbh,'UpdateGUI');||MCHP_ADC_SAME5x_Callback(gcbh,'UpdateGUI');||MCHP_ADC_SAME5x_Callback(gcbh,'UpdateGUI');||MCHP_ADC_SAME5x_Callback(gcbh,'UpdateGUI');||MCHP_ADC_SAME5x_Callback(gcbh,'UpdateGUI');||MCHP_ADC_SAME5x_Callback(gcbh,'UpdateGUI');||MCHP_ADC_SAME5x_Callback(gcbh,'UpdateGUI');||MCHP_ADC_SAME5x_Callback(gcbh,'UpdateGUI');||MCHP_ADC_SAME5x_Callback(gcbh,'UpdateGUI');||MCHP_ADC_SAME5x_Callback(gcbh,'UpdateGUI');||MCHP_ADC_SAME5x_Callback(gcbh,'UpdateGUI');||MCHP_ADC_SAME5x_Callback(gcbh,'UpdateGUI');||||||||MCHP_ADC_SAME5x_Callback(gcbh,'UpdateGUI');||MCHP_ADC_SAME5x_Callback(gcbh,'UpdateGUI');||MCHP_ADC_SAME5x_Callback(gcbh,'UpdateGUI');||MCHP_ADC_SAME5x_Callback(gcbh,'UpdateGUI');||MCHP_ADC_SAME5x_Callback(gcbh,'UpdateGUI');||MCHP_ADC_SAME5x_Callback(gcbh,'UpdateGUI');||MCHP_ADC_SAME5x_Callback(gcbh,'UpdateGUI');||MCHP_ADC_SAME5x_Callback(gcbh,'UpdateGUI');||MCHP_ADC_SAME5x_Callback(gcbh,'UpdateGUI');||MCHP_ADC_SAME5x_Callback(gcbh,'UpdateGUI');||MCHP_ADC_SAME5x_Callback(gcbh,'UpdateGUI');||MCHP_ADC_SAME5x_Callback(gcbh,'UpdateGUI');||||||||MCHP_ADC_SAME5x_Callback(gcbh,'UpdateGUI');||MCHP_ADC_SAME5x_Callback(gcbh,'UpdateGUI');||MCHP_ADC_SAME5x_Callback(gcbh,'UpdateGUI');||MCHP_ADC_SAME5x_Callback(gcbh,'UpdateGUI');||MCHP_ADC_SAME5x_Callback(gcbh,'UpdateGUI');||MCHP_ADC_SAME5x_Callback(gcbh,'UpdateGUI');||MCHP_ADC_SAME5x_Callback(gcbh,'UpdateGUI');||MCHP_ADC_SAME5x_Callback(gcbh,'UpdateGUI');||MCHP_ADC_SAME5x_Callback(gcbh,'UpdateGUI');||MCHP_ADC_SAME5x_Callback(gcbh,'UpdateGUI');||MCHP_ADC_SAME5x_Callback(gcbh,'UpdateGUI');||MCHP_ADC_SAME5x_Callback(gcbh,'UpdateGUI');|||||
      mask TabNameString: Main,Main,Main,Main,Main,Main,Main,Main,Seq 0,Seq 0,Seq 0,Seq 0,Seq 0,Seq 0,Seq 0,Seq 0,Seq 0,Seq 0,Seq 0,Seq 0,Seq 0,Seq 0,Seq 0,Seq 0,Seq 0,Seq 0,Seq 0,Seq 0,Seq 0,Seq 0,Seq 0,Seq 0,Seq 0,Seq 0,Seq 0,Seq 0,Seq 0,Seq 0,Seq 1,Seq 1,Seq 1,Seq 1,Seq 1,Seq 1,Seq 1,Seq 1,Seq 1,Seq 1,Seq 1,Seq 1,Seq 1,Seq 1,Seq 1,Seq 1,Seq 1,Seq 1,Seq 1,Seq 1,Seq 1,Seq 1,Seq 1,Seq 1,Seq 1,Seq 1,Seq 1,Seq 1,Seq 1,Seq 1,Seq 2,Seq 2,Seq 2,Seq 2,Seq 2,Seq 2,Seq 2,Seq 2,Seq 2,Seq 2,Seq 2,Seq 2,Seq 2,Seq 2,Seq 2,Seq 2,Seq 2,Seq 2,Seq 2,Seq 2,Seq 2,Seq 2,Seq 2,Seq 2,Seq 2,Seq 2,Seq 2,Seq 2,Seq 2,Seq 2,Seq 3,Seq 3,Seq 3,Seq 3,Seq 3,Seq 3,Seq 3,Seq 3,Seq 3,Seq 3,Seq 3,Seq 3,Seq 3,Seq 3,Seq 3,Seq 3,Seq 3,Seq 3,Seq 3,Seq 3,Seq 3,Seq 3,Seq 3,Seq 3,Seq 3,Seq 3,Seq 3,Seq 3,Seq 3,Seq 3,Seq 4,Seq 4,Seq 4,Seq 4,Seq 4,Seq 4,Seq 4,Seq 4,Seq 4,Seq 4,Seq 4,Seq 4,Seq 4,Seq 4,Seq 4,Seq 4,Seq 4,Seq 4,Seq 4,Seq 4,Seq 4,Seq 4,Seq 4,Seq 4,Seq 4,Seq 4,Seq 4,Seq 4,Seq 4,Seq 4,Seq 5,Seq 5,Seq 5,Seq 5,Seq 5,Seq 5,Seq 5,Seq 5,Seq 5,Seq 5,Seq 5,Seq 5,Seq 5,Seq 5,Seq 5,Seq 5,Seq 5,Seq 5,Seq 5,Seq 5,Seq 5,Seq 5,Seq 5,Seq 5,Seq 5,Seq 5,Seq 5,Seq 5,Seq 5,Seq 5
      mask Display:
      | MCHP_DrawLogo;fprintf('ADC SAM 5x');
      | port_label('output',1,'ADC0_AIN6');
      | port_label('output',2,'ADC1_AIN8');
  ADC SAMx7 : S-Function  Priority=-2000  LoadFcn=MCHP_Fun.Load_EvalIn_ws(gcbh);  InitFcn=MCHP_AFEC_SAM7x_Callback(gcbh,'InitFcn');  FunctionName=MCHP_AFEC_SAM7x  Parameters=MCHP_AFEC_SAM7x_Callback(gcbh,'S_INPUT'),MCHP_AFEC_SAM7x_Callback(gcbh,'S_OUTPUT'),MCHP_AFEC_SAM7x_Callback(gcbh,'S_INPUT_Size'),MCHP_AFEC_SAM7x_Callback(gcbh,'S_OUTPUT_Size'),MCHP_AFEC_SAM7x_Callback(gcbh,'S_ListCustomDatatype'),SampleTime,0  EnableBusSupport=off  mask(ADC for SAMx7){AFECx=AFE Controller 0, SIGNMODE_SingleEnded=Unsigned (uint16), SIGNMODE_Differential=Signed    (int16), AFEC0_seq0=Dynamic Options, AFEC0_seq0_TXT=AD0 / PD30, AFEC1_seq0=Dynamic Options, AFEC1_seq0_TXT=Temperature, AFEC0_seq1=Dynamic Options, AFEC0_seq1_TXT=Not used, AFEC1_seq1=Dynamic Options, AFEC1_seq1_TXT=Not used, AFEC0_seq2=Dynamic Options, AFEC0_seq2_TXT=Not used, AFEC1_seq2=Dynamic Options, AFEC1_seq2_TXT=Not used, AFEC0_seq3=Dynamic Options, AFEC0_seq3_TXT=Not used, AFEC1_seq3=Dynamic Options, AFEC1_seq3_TXT=Not used, AFEC0_seq4=Dynamic Options, AFEC0_seq4_TXT=Not used, AFEC1_seq4=Dynamic Options, AFEC1_seq4_TXT=Not used, AFEC0_seq5=Dynamic Options, AFEC0_seq5_TXT=Not used, AFEC1_seq5=Dynamic Options, AFEC1_seq5_TXT=Not used, AFEC0_seq6=Dynamic Options, AFEC0_seq6_TXT=Not used, AFEC1_seq6=Dynamic Options, AFEC1_seq6_TXT=Not used, AFEC0_seq7=Dynamic Options, AFEC0_seq7_TXT=Not used, AFEC1_seq7=Dynamic Options, AFEC1_seq7_TXT=Not used, AFEC0_seq8=Dynamic Options, AFEC0_seq8_TXT=Not used, AFEC1_seq8=Dynamic Options, AFEC1_seq8_TXT=Not used, AFEC0_seq9=Dynamic Options, AFEC0_seq9_TXT=Not used, AFEC1_seq9=Dynamic Options, AFEC1_seq9_TXT=Not used, AFEC0_seq10=Dynamic Options, AFEC0_seq10_TXT=Not used, AFEC1_seq10=Dynamic Options, AFEC1_seq10_TXT=Not used, AFEC0_seq11=Dynamic Options, AFEC0_seq11_TXT=Not used, AFEC1_seq11=Dynamic Options, AFEC1_seq11_TXT=Not used, SampleTime=.001, S_INPUT=[-1], S_INPUT_Size=[3], S_OUTPUT=[], S_OUTPUT_Size=[], S_ListCustomDatatype=S.S_ListCustomDatatype={};, evalin_ws=, MCHP_AFECC_CLOCK_REQUEST='', MCHP_AFECC_CLOCK_RESULT='', MCHP_USER_INTERRUPTS=0, MCHP_PORT=, MCHP_MASTERLINK=tpf02090e2_a548_4000_93a9_853b545f00d8_saveas/Microchip Master, Rin=< 200 Ohm, RES=12-bit Standard, AFEC0_Synchronisation=Triggered by user defined source, AFEC0_Trig=PWM0 event line 0, AFEC0_TrigTimeStep=on, AFEC1_Synchronisation=Triggered at end of previous time step, AFEC1_Trig=AFE1_ADTRG input pin, AFEC1_TrigTimeStep=on, ADC_TrigInfo=0, AFEC0_seq0_GAIN=1, AFEC1_seq0_GAIN=1, AFEC0_seq1_GAIN=1, AFEC1_seq1_GAIN=1, AFEC0_seq2_GAIN=1, AFEC1_seq2_GAIN=1, AFEC0_seq3_GAIN=1, AFEC1_seq3_GAIN=1, AFEC0_seq4_GAIN=1, AFEC1_seq4_GAIN=1, AFEC0_seq5_GAIN=1, AFEC1_seq5_GAIN=1, AFEC0_seq6_GAIN=1, AFEC1_seq6_GAIN=1, AFEC0_seq7_GAIN=1, AFEC1_seq7_GAIN=1, AFEC0_seq8_GAIN=1, AFEC1_seq8_GAIN=1, AFEC0_seq9_GAIN=1, AFEC1_seq9_GAIN=1, AFEC0_seq10_GAIN=1, AFEC1_seq10_GAIN=1, AFEC0_seq11_GAIN=1, AFEC1_seq11_GAIN=1, AFEC0_seq0_OFFSET=0, AFEC1_seq0_OFFSET=0, AFEC0_seq1_OFFSET=0, AFEC1_seq1_OFFSET=0, AFEC0_seq2_OFFSET=0, AFEC1_seq2_OFFSET=0, AFEC0_seq3_OFFSET=0, AFEC1_seq3_OFFSET=0, AFEC0_seq4_OFFSET=0, AFEC1_seq4_OFFSET=0, AFEC0_seq5_OFFSET=0, AFEC1_seq5_OFFSET=0, AFEC0_seq6_OFFSET=0, AFEC1_seq6_OFFSET=0, AFEC0_seq7_OFFSET=0, AFEC1_seq7_OFFSET=0, AFEC0_seq8_OFFSET=0, AFEC1_seq8_OFFSET=0, AFEC0_seq9_OFFSET=0, AFEC1_seq9_OFFSET=0, AFEC0_seq10_OFFSET=0, AFEC1_seq10_OFFSET=0, AFEC0_seq11_OFFSET=0, AFEC1_seq11_OFFSET=0}
      mask prompts: AFECx "Select ADC (AFEC) Controller :"; SIGNMODE_SingleEnded "Single-Ended conversion output are"; SIGNMODE_Differential "Differential conversions output are"; AFEC0_seq0 "AFEC0 seq 0"; AFEC0_seq0_TXT "sequence x"; AFEC1_seq0 "AFEC1 seq 0"; AFEC1_seq0_TXT "sequence x"; AFEC0_seq1 "AFEC0 seq 1"; AFEC0_seq1_TXT "sequence x"; AFEC1_seq1 "AFEC1 seq 1"; AFEC1_seq1_TXT "sequence x"; AFEC0_seq2 "AFEC0 seq 2"; AFEC0_seq2_TXT "sequence x"; AFEC1_seq2 "AFEC1 seq 2"; AFEC1_seq2_TXT "sequence x"; AFEC0_seq3 "AFEC0 seq 3"; AFEC0_seq3_TXT "sequence x"; AFEC1_seq3 "AFEC1 seq 3"; AFEC1_seq3_TXT "sequence x"; AFEC0_seq4 "AFEC0 seq 4"; AFEC0_seq4_TXT "sequence x"; AFEC1_seq4 "AFEC1 seq 4"; AFEC1_seq4_TXT "sequence x"; AFEC0_seq5 "AFEC0 seq 5"; AFEC0_seq5_TXT "sequence x"; AFEC1_seq5 "AFEC1 seq 5"; AFEC1_seq5_TXT "sequence x"; AFEC0_seq6 "AFEC0 seq 6"; AFEC0_seq6_TXT "sequence x"; AFEC1_seq6 "AFEC1 seq 6"; AFEC1_seq6_TXT "sequence x"; AFEC0_seq7 "AFEC0 seq 7"; AFEC0_seq7_TXT "sequence x"; AFEC1_seq7 "AFEC1 seq 7"; AFEC1_seq7_TXT "sequence x"; AFEC0_seq8 "AFEC0 seq 8"; AFEC0_seq8_TXT "sequence x"; AFEC1_seq8 "AFEC1 seq 8"; AFEC1_seq8_TXT "sequence x"; AFEC0_seq9 "AFEC0 seq 9"; AFEC0_seq9_TXT "sequence x"; AFEC1_seq9 "AFEC1 seq 9"; AFEC1_seq9_TXT "sequence x"; AFEC0_seq10 "AFEC0 seq 10"; AFEC0_seq10_TXT "sequence x"; AFEC1_seq10 "AFEC1 seq 10"; AFEC1_seq10_TXT "sequence x"; AFEC0_seq11 "AFEC0 seq 11"; AFEC0_seq11_TXT "sequence x"; AFEC1_seq11 "AFEC1 seq 11"; AFEC1_seq11_TXT "sequence x"; SampleTime "Block output sample time"; Rin "Input impedance / minimum Sample time"; RES "Resolution and Digital Filter"; AFEC0_Synchronisation "AFEC0 sequence is"; AFEC0_Trig "User defined trigger (AFEC0):"; AFEC0_TrigTimeStep "The model base Time Step is triggered by AFEC0 last seq conversion"; AFEC1_Synchronisation "AFEC1 sequence is"; AFEC1_Trig "User defined trigger (AFEC1):"; AFEC1_TrigTimeStep "The model base Time Step is triggered by AFEC1 last seq conversion"; ADC_TrigInfo "ADC Trigger Info"; AFEC0_seq0_GAIN "AD0 - PD30 Gain"; AFEC1_seq0_GAIN "AD0 - PB1 Gain"; AFEC0_seq1_GAIN "AD1 - PA21 Gain"; AFEC1_seq1_GAIN "AD1 - PC13 Gain"; AFEC0_seq2_GAIN "AD2 - PB3 Gain"; AFEC1_seq2_GAIN "AD2 - PC15 Gain"; AFEC0_seq3_GAIN "AD3 - PE5 Gain"; AFEC1_seq3_GAIN "AD3 - PC12 Gain"; AFEC0_seq4_GAIN "AD4 - PE4 Gain"; AFEC1_seq4_GAIN "AD4 - PC29 Gain"; AFEC0_seq5_GAIN "AD5 - PB2 Gain"; AFEC1_seq5_GAIN "AD5 - PC30 Gain"; AFEC0_seq6_GAIN "AD6 - PA17 Gain"; AFEC1_seq6_GAIN "AD6 - PC31 Gain"; AFEC0_seq7_GAIN "AD7 - PA18 Gain"; AFEC1_seq7_GAIN "AD7 - PC26 Gain"; AFEC0_seq8_GAIN "AD8 - PA19 Gain"; AFEC1_seq8_GAIN "AD8 - PC27 Gain"; AFEC0_seq9_GAIN "AD9 - PA20 Gain"; AFEC1_seq9_GAIN "AD9 - PC0 Gain"; AFEC0_seq10_GAIN "AD10 - PB0 Gain"; AFEC1_seq10_GAIN "AD10 - PE3 Gain"; AFEC0_seq11_GAIN "AD11 - AFEC0 Gain"; AFEC1_seq11_GAIN "AD11 - AFEC1 Gain"; AFEC0_seq0_OFFSET "AD0 - PD30 Offset within [-512 511]"; AFEC1_seq0_OFFSET "AD0 - PB1 Offset within [-512 511]"; AFEC0_seq1_OFFSET "AD1 - PA21 Offset within [-512 511]"; AFEC1_seq1_OFFSET "AD1 - PC13 Offset within [-512 511]"; AFEC0_seq2_OFFSET "AD2 - PB3 Offset within [-512 511]"; AFEC1_seq2_OFFSET "AD2 - PC15 Offset within [-512 511]"; AFEC0_seq3_OFFSET "AD3 - PE5 Offset within [-512 511]"; AFEC1_seq3_OFFSET "AD3 - PC12 Offset within [-512 511]"; AFEC0_seq4_OFFSET "AD4 - PE4 Offset within [-512 511]"; AFEC1_seq4_OFFSET "AD4 - PC29 Offset within [-512 511]"; AFEC0_seq5_OFFSET "AD5 - PB2 Offset within [-512 511]"; AFEC1_seq5_OFFSET "AD5 - PC30 Offset within [-512 511]"; AFEC0_seq6_OFFSET "AD6 - PA17 Offset within [-512 511]"; AFEC1_seq6_OFFSET "AD6 - PC31 Offset within [-512 511]"; AFEC0_seq7_OFFSET "AD7 - PA18 Offset within [-512 511]"; AFEC1_seq7_OFFSET "AD7 - PC26 Offset within [-512 511]"; AFEC0_seq8_OFFSET "AD8 - PA19 Offset within [-512 511]"; AFEC1_seq8_OFFSET "AD8 - PC27 Offset within [-512 511]"; AFEC0_seq9_OFFSET "AD9 - PA20 Offset within [-512 511]"; AFEC1_seq9_OFFSET "AD9 - PC0 Offset within [-512 511]"; AFEC0_seq10_OFFSET "AD10 - PB0 Offset within [-512 511]"; AFEC1_seq10_OFFSET "AD10 - PE3 Offset within [-512 511]"; AFEC0_seq11_OFFSET "AD11 - AFEC0 Offset within [-512 511]"; AFEC1_seq11_OFFSET "AD11 - AFEC1 Offset within [-512 511]"
      mask help:
      | Configure the Analog Front End Controller (AFEC).
      |
      | Two AFEC modules can be configured independantly using two ADC blocks.
      | They will have common parameters when set with one common block.
      |
      | The 11 analog input pins are different for each AFEC.
      |
      | The sequence set in the block is listed in sampling chronological order.
      mask init:
      | MCHP_AFEC_SAM7x_Callback(gcbh,'INITIALISATION');
      settings: CopyFcn=MCHP_AFEC_SAM7x_Callback(gcbh,'CopyFcn');  PreSaveFcn=MCHP_Fun.PreSaveFcn_DynamicOptions(gcbh);  OpenFcn=MCHP_AFEC_SAM7x_Callback(gcbh,'OPEN');
      mask StyleString: popup(AFE Controller 0|AFE Controller 1|AFE Controller 0 & 1),popup(Unsigned (uint16)|Signed    (int16)),popup(Unsigned (uint16)|Signed    (int16)),popup(Dynamic Options),edit,popup(Dynamic Options),edit,popup(Dynamic Options),edit,popup(Dynamic Options),edit,popup(Dynamic Options),edit,popup(Dynamic Options),edit,popup(Dynamic Options),edit,popup(Dynamic Options),edit,popup(Dynamic Options),edit,popup(Dynamic Options),edit,popup(Dynamic Options),edit,popup(Dynamic Options),edit,popup(Dynamic Options),edit,popup(Dynamic Options),edit,popup(Dynamic Options),edit,popup(Dynamic Options),edit,popup(Dynamic Options),edit,popup(Dynamic Options),edit,popup(Dynamic Options),edit,popup(Dynamic Options),edit,popup(Dynamic Options),edit,popup(Dynamic Options),edit,popup(Dynamic Options),edit,popup(Dynamic Options),edit,edit,edit,edit,edit,edit,edit,edit,edit,edit,edit,edit,edit,popup(< 200 Ohm|< 500 Ohm|< 1    kOhm|< 2    kOhm|< 5    kOhm|< 10   kOhm|< 20   kOhm|< 50   kOhm|< 100  kOhm|< 200  kOhm|< 500  kOhm|max sampling time),popup(10-bit Low Resolution|12-bit Standard|13-bit (Average 4 conversions)|14-bit (Average 16 conversions)|15-bit (Average 64 conversions)|16-bit (Average 256 conversions)),popup(Triggered at end of previous time step|Software triggered after reading last converted value|Triggered by user defined source|Free Run. Output is last converted value),popup(AFE0_ADTRG input pin|PWM0 event line 0|PWM0 event line 1|Timer Counter Channel 0|Timer Counter Channel 1|Timer Counter Channel 2|Analog Comparator),checkbox,popup(Triggered at end of previous time step|Software triggered after reading last converted value|Triggered by user defined source|Free Run. Output is last converted value),popup(AFE1_ADTRG input pin|PWM1 event line 0|PWM1 event line 1|Timer Counter Channel 3|Timer Counter Channel 4|Timer Counter Channel 5|Analog Comparator),checkbox,edit,popup(1|2|4),popup(1|2|4),popup(1|2|4),popup(1|2|4),popup(1|2|4),popup(1|2|4),popup(1|2|4),popup(1|2|4),popup(1|2|4),popup(1|2|4),popup(1|2|4),popup(1|2|4),popup(1|2|4),popup(1|2|4),popup(1|2|4),popup(1|2|4),popup(1|2|4),popup(1|2|4),popup(1|2|4),popup(1|2|4),popup(1|2|4),popup(1|2|4),popup(1|2|4),popup(1|2|4),edit,edit,edit,edit,edit,edit,edit,edit,edit,edit,edit,edit,edit,edit,edit,edit,edit,edit,edit,edit,edit,edit,edit,edit
      mask CallbackString: MCHP_AFEC_SAM7x_Callback(gcbh,'UpdateGUI');|||MCHP_AFEC_SAM7x_Callback(gcbh,'UpdateGUI');|MCHP_AFEC_SAM7x_Callback(gcbh,'UpdateGUI');|MCHP_AFEC_SAM7x_Callback(gcbh,'UpdateGUI');|MCHP_AFEC_SAM7x_Callback(gcbh,'UpdateGUI');|MCHP_AFEC_SAM7x_Callback(gcbh,'UpdateGUI');|MCHP_AFEC_SAM7x_Callback(gcbh,'UpdateGUI');|MCHP_AFEC_SAM7x_Callback(gcbh,'UpdateGUI');|MCHP_AFEC_SAM7x_Callback(gcbh,'UpdateGUI');||MCHP_AFEC_SAM7x_Callback(gcbh,'UpdateGUI');||MCHP_AFEC_SAM7x_Callback(gcbh,'UpdateGUI');|MCHP_AFEC_SAM7x_Callback(gcbh,'UpdateGUI');|MCHP_AFEC_SAM7x_Callback(gcbh,'UpdateGUI');|MCHP_AFEC_SAM7x_Callback(gcbh,'UpdateGUI');|MCHP_AFEC_SAM7x_Callback(gcbh,'UpdateGUI');|MCHP_AFEC_SAM7x_Callback(gcbh,'UpdateGUI');|MCHP_AFEC_SAM7x_Callback(gcbh,'UpdateGUI');|MCHP_AFEC_SAM7x_Callback(gcbh,'UpdateGUI');|MCHP_AFEC_SAM7x_Callback(gcbh,'UpdateGUI');|MCHP_AFEC_SAM7x_Callback(gcbh,'UpdateGUI');|MCHP_AFEC_SAM7x_Callback(gcbh,'UpdateGUI');|MCHP_AFEC_SAM7x_Callback(gcbh,'UpdateGUI');|MCHP_AFEC_SAM7x_Callback(gcbh,'UpdateGUI');|MCHP_AFEC_SAM7x_Callback(gcbh,'UpdateGUI');|MCHP_AFEC_SAM7x_Callback(gcbh,'UpdateGUI');|MCHP_AFEC_SAM7x_Callback(gcbh,'UpdateGUI');|MCHP_AFEC_SAM7x_Callback(gcbh,'UpdateGUI');|MCHP_AFEC_SAM7x_Callback(gcbh,'UpdateGUI');|MCHP_AFEC_SAM7x_Callback(gcbh,'UpdateGUI');|MCHP_AFEC_SAM7x_Callback(gcbh,'UpdateGUI');|MCHP_AFEC_SAM7x_Callback(gcbh,'UpdateGUI');|MCHP_AFEC_SAM7x_Callback(gcbh,'UpdateGUI');|MCHP_AFEC_SAM7x_Callback(gcbh,'UpdateGUI');|MCHP_AFEC_SAM7x_Callback(gcbh,'UpdateGUI');|MCHP_AFEC_SAM7x_Callback(gcbh,'UpdateGUI');|MCHP_AFEC_SAM7x_Callback(gcbh,'UpdateGUI');|MCHP_AFEC_SAM7x_Callback(gcbh,'UpdateGUI');|MCHP_AFEC_SAM7x_Callback(gcbh,'UpdateGUI');|MCHP_AFEC_SAM7x_Callback(gcbh,'UpdateGUI');|MCHP_AFEC_SAM7x_Callback(gcbh,'UpdateGUI');|MCHP_AFEC_SAM7x_Callback(gcbh,'UpdateGUI');|MCHP_AFEC_SAM7x_Callback(gcbh,'UpdateGUI');|MCHP_AFEC_SAM7x_Callback(gcbh,'UpdateGUI');|MCHP_AFEC_SAM7x_Callback(gcbh,'UpdateGUI');|MCHP_AFEC_SAM7x_Callback(gcbh,'UpdateGUI');|MCHP_AFEC_SAM7x_Callback(gcbh,'UpdateGUI');|MCHP_AFEC_SAM7x_Callback(gcbh,'UpdateGUI');|||||||||||||||MCHP_AFEC_SAM7x_Callback(gcbh,'UpdateGUI');|||MCHP_AFEC_SAM7x_Callback(gcbh,'UpdateGUI');|||||||||||||||||||||||||||||||||||||||||||||||||||
      mask TabNameString: Analog Channels,Analog Channels,Analog Channels,Analog Channels,Analog Channels,Analog Channels,Analog Channels,Analog Channels,Analog Channels,Analog Channels,Analog Channels,Analog Channels,Analog Channels,Analog Channels,Analog Channels,Analog Channels,Analog Channels,Analog Channels,Analog Channels,Analog Channels,Analog Channels,Analog Channels,Analog Channels,Analog Channels,Analog Channels,Analog Channels,Analog Channels,Analog Channels,Analog Channels,Analog Channels,Analog Channels,Analog Channels,Analog Channels,Analog Channels,Analog Channels,Analog Channels,Analog Channels,Analog Channels,Analog Channels,Analog Channels,Analog Channels,Analog Channels,Analog Channels,Analog Channels,Analog Channels,Analog Channels,Analog Channels,Analog Channels,Analog Channels,Analog Channels,Analog Channels,Analog Channels,Analog Channels,Analog Channels,Analog Channels,Analog Channels,Analog Channels,Analog Channels,Analog Channels,Analog Channels,Analog Channels,Analog Channels,Analog Channels,Options,Options,Options,Options,Options,Options,Options,Options,Options,Gain,Gain,Gain,Gain,Gain,Gain,Gain,Gain,Gain,Gain,Gain,Gain,Gain,Gain,Gain,Gain,Gain,Gain,Gain,Gain,Gain,Gain,Gain,Gain,Offset,Offset,Offset,Offset,Offset,Offset,Offset,Offset,Offset,Offset,Offset,Offset,Offset,Offset,Offset,Offset,Offset,Offset,Offset,Offset,Offset,Offset,Offset,Offset
      mask Display:
      | fprintf(['AFEC SAMx7\n' AFECx(4:end)]);
      | port_label('output',1,'PD30');
  ADC dsPIC High Speed SAR : S-Function  InitFcn=MCHP_ADC_HighSpeed_SAR_dsPIC_Callback(gcbh,'InitFcn');  FunctionName=MCHP_ADC_HighSpeed_SAR_dsPIC  Parameters=MCHP_ADC_HighSpeed_SAR_dsPIC_Callback(gcbh,'S_INPUT'),MCHP_ADC_HighSpeed_SAR_dsPIC_Callback(gcbh,'S_OUTPUT'),MCHP_ADC_HighSpeed_SAR_dsPIC_Callback(gcbh,'S_INPUT_Size'),MCHP_ADC_HighSpeed_SAR_dsPIC_Callback(gcbh,'S_OUTPUT_Size'),MCHP_ADC_HighSpeed_SAR_dsPIC_Callback(gcbh,'S_ListCustomDatatype'),SampleTime,0  EnableBusSupport=off  mask(ADC SAR for dsPIC EP GS family){ACLKCON=Optimized for PWM resolution & ADC conversion speed, ADC_FRACT=Integer (right aligned), ADC_NRE=off, DMA_Size=Single trigger - (default), ADC_Synchronisation=Triggered at end of previous time step, ADC_Trig=Dynamic Options, ADC_Trig_TXT=Timer2 period match, ADC_TrigTimeStep=Trig model step after all sample using this trigger are converted, ADC_TrigInfo=0, SampleTime=.001, S_INPUT=[], S_INPUT_Size=[], S_OUTPUT=[5  5], S_OUTPUT_Size=[1  1], S_ListCustomDatatype=S.S_ListCustomDatatype={};, MCHP_USER_INTERRUPTS={ADCAN0}{ADCBUF0}{ADC Data 0 Ready}{VectorName(ADCAN0Interrupt) Priority(-1) RegisterReadClear(ADCBUF0)Config_BitSet(ADIELbits.IE0) };, MCHP_PORT={Analog Input 0}{AN0}15:2:A0;, MCHP_MASTERLINK=Dvpt_33EP64GS504_ADC_ExportLib/Microchip Master, MCHP_CRC=3588008, ADC_Info=Total Time = 279.412(ns), ADC0_pin=Dynamic Options, ADC0_pin_TXT=AN0 / A0 / Pin[21], ADC0_R=< 10   kOhm, ADC0_res=12 bits, ADC0_signed=signed 16 bits, ADC0_FILTER=No Oversampling, ADC0_FILTER_nSamples=256 samples, ADC0_STRGEN=End sampling and start conversion, ADC0_STRGEN_on=Start sampling followed by conversion, ADC0_SSAMPEN=off, ADC0_Info=tSmp_min=338.24(ns) x 0 = 0(s) ; tConv=272.06(ns) x 1 = 272.06(ns) ; TOTAL=279.41(ns), ADC1_pin=Dynamic Options, ADC1_pin_TXT=Not used, ADC1_R=< 200 Ohm, ADC1_res=12 bits, ADC1_signed=signed 16 bits, ADC1_FILTER=No Oversampling, ADC1_FILTER_nSamples=128 samples, ADC1_STRGEN=End sampling and start conversion, ADC1_STRGEN_on=Start sampling followed by conversion, ADC1_SSAMPEN=off, ADC1_Info=tSmp_min=14.706(ns) x 0 = 0(s) ; tConv=154.41(ns) x 0 = 0(s) ; TOTAL=0(s), ADC2_pin=Dynamic Options, ADC2_pin_TXT=Not used, ADC2_R=< 5    kOhm, ADC2_res=12 bits, ADC2_signed=signed 16 bits, ADC2_FILTER=No Oversampling, ADC2_FILTER_nSamples=256 samples, ADC2_STRGEN=End sampling and start conversion, ADC2_STRGEN_on=Start sampling followed by conversion, ADC2_SSAMPEN=on, ADC2_Info=tSmp_min=14.706(ns) x 0 = 0(s) ; tConv=154.41(ns) x 0 = 0(s) ; TOTAL=0(s), ADC3_pin=Dynamic Options, ADC3_pin_TXT=Not used, ADC3_R=< 10   kOhm, ADC3_res=12 bits, ADC3_signed=signed 16 bits, ADC3_FILTER=Burst convert of n samples are Summed, ADC3_FILTER_nSamples=64 samples, ADC3_STRGEN=End sampling and start conversion, ADC3_STRGEN_on=Start sampling followed by conversion, ADC3_SSAMPEN=on, ADC3_Info=tSmp_min=14.706(ns) x 0 = 0(s) ; tConv=154.41(ns) x 0 = 0(s) ; TOTAL=0(s), ADC4_pin=Dynamic Options, ADC4_pin_TXT=Not used, ADC4_R=< 200 Ohm, ADC4_res=12 bits, ADC4_signed=unsigned 16 bits, ADC4_FILTER=No Oversampling, ADC4_FILTER_nSamples=256 samples, ADC4_STRGEN=End sampling and start conversion, ADC4_STRGEN_on=Start sampling followed by conversion, ADC4_SSAMPEN=off, ADC4_Info=tSmp_min=14.706(ns) x 0 = 0(s) ; tConv=154.41(ns) x 0 = 0(s) ; TOTAL=0(s), ADC5_pin=Dynamic Options, ADC5_pin_TXT=Not used, ADC5_R=< 200 Ohm, ADC5_res=12 bits, ADC5_signed=unsigned 16 bits, ADC5_FILTER=Burst convert of n samples are Summed, ADC5_FILTER_nSamples=256 samples, ADC5_STRGEN=End sampling and start conversion, ADC5_STRGEN_on=Start sampling followed by conversion, ADC5_SSAMPEN=on, ADC5_Info=tSmp_min=14.706(ns) x 0 = 0(s) ; tConv=154.41(ns) x 0 = 0(s) ; TOTAL=0(s), ADC6_pin=Dynamic Options, ADC6_pin_TXT=Not used, ADC6_R=< 200 Ohm, ADC6_res=12 bits, ADC6_signed=unsigned 16 bits, ADC6_FILTER=Burst convert of n samples are Summed, ADC6_FILTER_nSamples=256 samples, ADC6_STRGEN=End sampling and start conversion, ADC6_STRGEN_on=Start sampling followed by conversion, ADC6_SSAMPEN=on, ADC6_Info=tSmp_min=14.706(ns) x 0 = 0(s) ; tConv=154.41(ns) x 0 = 0(s) ; TOTAL=0(s), ADC7_R=< 10   kOhm, ADC7_res=12 bits, ADC7_AN0=Not used, ADC7_AN1=Not used, ADC7_AN2=Not used, ADC7_AN3=Not used, ADC7_AN4=Not used, ADC7_AN5=Not used, ADC7_AN6=Not used, ADC7_AN7=Not used, ADC7_AN8=Not used, ADC7_AN9=Not used, ADC7_AN10=Not used, ADC7_AN11=Not used, ADC7_AN12=Not used, ADC7_AN13=Not used, ADC7_AN14=Not used, ADC7_AN15=Not used, ADC7_AN16=Not used, ADC7_AN17=Not used, ADC7_AN18=Not used, ADC7_AN19=Not used, ADC7_AN20=Not used, ADC7_AN21=Not used, ADC7_AN22=Not used, ADC7_AN23=Not used, ADC7_AN24=Not used, ADC7_AN25=Not used, ADC7_AN26=Not used, ADC7_AN27=Not used, ADC7_AN28=Not used, ADC7_AN29=Not used, ADC7_AN30=Not used, ADC7_AN31=Not used, IVref=Not used, IVTemp=Not used, ADC7_Info=tSmp_min=14.706(ns) x 0 = 0(s) ; tConv=154.41(ns) x 0 = 0(s) ; TOTAL=0(s)}
